simulink model "s_c_nbe_m32k"  (R2016b)
settings: Solver=VariableStepDiscrete  StartTime=0.0  StopTime=2^(fft_stages)*10  RelTol=1e-3
undefined symbols (not defined in the file or in its folder): fft_stages, n_taps, output_bits, xengbits
undefined symbols (not defined in the file): Coeffs, pfb_coeff_gen_calc
libraries: xbsIndex_r4 x12104, xps_library x3, casper_library_delays x2, casper_library_misc x1
(part 21 of 104)

== system s_c_nbe_m32k/DDC/dec_fir_async ==
  sync_in : Inport
  dv_in : Inport  Port=2
  real1 : Inport  Port=3
  imag1 : Inport  Port=4
  real2 : Inport  Port=5
  imag2 : Inport  Port=6
  real3 : Inport  Port=7
  imag3 : Inport  Port=8
  real4 : Inport  Port=9
  imag4 : Inport  Port=10
  real5 : Inport  Port=11
  imag5 : Inport  Port=12
  real6 : Inport  Port=13
  imag6 : Inport  Port=14
  real7 : Inport  Port=15
  imag7 : Inport  Port=16
  real8 : Inport  Port=17
  imag8 : Inport  Port=18
  convert1 : xbsIndex_r4/Convert  gui_display_data_type=Fixed-point  arith_type="Signed  (2's comp)"  n_bits=25  bin_pt=24  float_type=Single  exp_bits=8  fraction_bits=24  quantization="Round  (unbiased: +/- Inf)"  overflow=Wrap  en=off  latency=2  pipeline=off  dbl_ovrd=off  block_type=convert
  convert2 : xbsIndex_r4/Convert  gui_display_data_type=Fixed-point  arith_type="Signed  (2's comp)"  n_bits=25  bin_pt=24  float_type=Single  exp_bits=8  fraction_bits=24  quantization="Round  (unbiased: +/- Inf)"  overflow=Wrap  en=off  latency=2  pipeline=off  dbl_ovrd=off  block_type=convert
  dv_delay : xbsIndex_r4/Delay  rst=off  infoeditControl=Selection of Reset will increase slice count due to use of real FFs and instead of SRLs  en=off  latency=13  reg_retiming=off  dbl_ovrd=off  block_type=delay
      settings: infoedit=Hardware notes: A delay line is a chain, each link of which is an SRL16 or SRL32 followed by a flip-flop.
  fir_col_async1 : Subsystem  AncestorBlock=casper_library_downconverter/fir_col_async  mask(fir_col_async){n_inputs=8, coeff=[0.00099428  0.00087065  0.00071858  0.00055833  0.00040616  0.00027356  0.00016693   0.0001122], add_latency=1, mult_latency=2, coeff_bit_width=25, coeff_bin_pt=24, first_stage_hdl=on, adder_imp=DSP48, async=on, bus_input=off, input_width=0, input_bp=0, input_type=Signed, dbl=on}
      mask prompts: n_inputs "Inputs"; coeff "Coefficients"; add_latency "Add latency"; mult_latency "Mult Latency"; coeff_bit_width "Coefficient bit width"; coeff_bin_pt "Coefficient binary point"; first_stage_hdl "Implement first stage of adder trees on output as behavioural HDL"; adder_imp "Adder implementation"; async "Asynchronous ops"; bus_input "Bus input"; input_width "Input bitwidth"; input_bp "Input binary point"; input_type "Input datatype"; dbl "Double col"
      mask init:
      | fir_col_async_init(gcb);
      mask Help: eval('xlWeb(''http://casper.berkeley.edu/wiki/Fir_col'')')
      mask TypeOptions adder_imp: Behavioral | Fabric | DSP48
      mask Callback bus_input:
      | onoff = get_param(gcb, 'bus_input');
      | set_param_state(gcb, 'input_width', onoff)
      | set_param_state(gcb, 'input_bp', onoff)
      | set_param_state(gcb, 'input_type', onoff)
      mask TypeOptions input_type: Signed | Unsigned
  fir_col_async10 : Subsystem  AncestorBlock=casper_library_downconverter/fir_col_async  mask(fir_col_async){n_inputs=8, coeff=[0.0010344  0.00087109  0.00057317  0.00018922 -0.00021959 -0.00058921  -0.0008627  -0.0009989], add_latency=1, mult_latency=2, coeff_bit_width=25, coeff_bin_pt=24, first_stage_hdl=on, adder_imp=DSP48, async=on, bus_input=off, input_width=0, input_bp=0, input_type=Signed, dbl=on}
      mask prompts: n_inputs "Inputs"; coeff "Coefficients"; add_latency "Add latency"; mult_latency "Mult Latency"; coeff_bit_width "Coefficient bit width"; coeff_bin_pt "Coefficient binary point"; first_stage_hdl "Implement first stage of adder trees on output as behavioural HDL"; adder_imp "Adder implementation"; async "Asynchronous ops"; bus_input "Bus input"; input_width "Input bitwidth"; input_bp "Input binary point"; input_type "Input datatype"; dbl "Double col"
      mask init:
      | fir_col_async_init(gcb);
      mask Help: eval('xlWeb(''http://casper.berkeley.edu/wiki/Fir_col'')')
      mask TypeOptions adder_imp: Behavioral | Fabric | DSP48
      mask Callback bus_input:
      | onoff = get_param(gcb, 'bus_input');
      | set_param_state(gcb, 'input_width', onoff)
      | set_param_state(gcb, 'input_bp', onoff)
      | set_param_state(gcb, 'input_type', onoff)
      mask TypeOptions input_type: Signed | Unsigned
  fir_col_async11 : Subsystem  AncestorBlock=casper_library_downconverter/fir_col_async  mask(fir_col_async){n_inputs=8, coeff=[-0.0011284 -0.00097771 -0.00067706 -0.00027629     0.00016  0.00056292  0.00087004    0.001035], add_latency=1, mult_latency=2, coeff_bit_width=25, coeff_bin_pt=24, first_stage_hdl=on, adder_imp=DSP48, async=on, bus_input=off, input_width=0, input_bp=0, input_type=Signed, dbl=on}
      mask prompts: n_inputs "Inputs"; coeff "Coefficients"; add_latency "Add latency"; mult_latency "Mult Latency"; coeff_bit_width "Coefficient bit width"; coeff_bin_pt "Coefficient binary point"; first_stage_hdl "Implement first stage of adder trees on output as behavioural HDL"; adder_imp "Adder implementation"; async "Asynchronous ops"; bus_input "Bus input"; input_width "Input bitwidth"; input_bp "Input binary point"; input_type "Input datatype"; dbl "Double col"
      mask init:
      | fir_col_async_init(gcb);
      mask Help: eval('xlWeb(''http://casper.berkeley.edu/wiki/Fir_col'')')
      mask TypeOptions adder_imp: Behavioral | Fabric | DSP48
      mask Callback bus_input:
      | onoff = get_param(gcb, 'bus_input');
      | set_param_state(gcb, 'input_width', onoff)
      | set_param_state(gcb, 'input_bp', onoff)
      | set_param_state(gcb, 'input_type', onoff)
      mask TypeOptions input_type: Signed | Unsigned
  fir_col_async12 : Subsystem  AncestorBlock=casper_library_downconverter/fir_col_async  mask(fir_col_async){n_inputs=8, coeff=[0.0012278   0.0010924  0.00078831  0.00036676 -0.00010386  -0.0005489 -0.00089924   -0.001102], add_latency=1, mult_latency=2, coeff_bit_width=25, coeff_bin_pt=24, first_stage_hdl=on, adder_imp=DSP48, async=on, bus_input=off, input_width=0, input_bp=0, input_type=Signed, dbl=on}
      mask prompts: n_inputs "Inputs"; coeff "Coefficients"; add_latency "Add latency"; mult_latency "Mult Latency"; coeff_bit_width "Coefficient bit width"; coeff_bin_pt "Coefficient binary point"; first_stage_hdl "Implement first stage of adder trees on output as behavioural HDL"; adder_imp "Adder implementation"; async "Asynchronous ops"; bus_input "Bus input"; input_width "Input bitwidth"; input_bp "Input binary point"; input_type "Input datatype"; dbl "Double col"
      mask init:
      | fir_col_async_init(gcb);
      mask Help: eval('xlWeb(''http://casper.berkeley.edu/wiki/Fir_col'')')
      mask TypeOptions adder_imp: Behavioral | Fabric | DSP48
      mask Callback bus_input:
      | onoff = get_param(gcb, 'bus_input');
      | set_param_state(gcb, 'input_width', onoff)
      | set_param_state(gcb, 'input_bp', onoff)
      | set_param_state(gcb, 'input_type', onoff)
      mask TypeOptions input_type: Signed | Unsigned
  fir_col_async13 : Subsystem  AncestorBlock=casper_library_downconverter/fir_col_async  mask(fir_col_async){n_inputs=8, coeff=[-0.0013452  -0.0012298 -0.00092426 -0.00048074  2.8225e-05  0.00052148  0.00092209   0.0011693], add_latency=1, mult_latency=2, coeff_bit_width=25, coeff_bin_pt=24, first_stage_hdl=on, adder_imp=DSP48, async=on, bus_input=off, input_width=0, input_bp=0, input_type=Signed, dbl=on}
      mask prompts: n_inputs "Inputs"; coeff "Coefficients"; add_latency "Add latency"; mult_latency "Mult Latency"; coeff_bit_width "Coefficient bit width"; coeff_bin_pt "Coefficient binary point"; first_stage_hdl "Implement first stage of adder trees on output as behavioural HDL"; adder_imp "Adder implementation"; async "Asynchronous ops"; bus_input "Bus input"; input_width "Input bitwidth"; input_bp "Input binary point"; input_type "Input datatype"; dbl "Double col"
      mask init:
      | fir_col_async_init(gcb);
      mask Help: eval('xlWeb(''http://casper.berkeley.edu/wiki/Fir_col'')')
      mask TypeOptions adder_imp: Behavioral | Fabric | DSP48
      mask Callback bus_input:
      | onoff = get_param(gcb, 'bus_input');
      | set_param_state(gcb, 'input_width', onoff)
      | set_param_state(gcb, 'input_bp', onoff)
      | set_param_state(gcb, 'input_type', onoff)
      mask TypeOptions input_type: Signed | Unsigned
  fir_col_async14 : Subsystem  AncestorBlock=casper_library_downconverter/fir_col_async  mask(fir_col_async){n_inputs=8, coeff=[0.0014712   0.0013813   0.0010768  0.00061055  5.9232e-05 -0.00048875 -0.00094762  -0.0012475], add_latency=1, mult_latency=2, coeff_bit_width=25, coeff_bin_pt=24, first_stage_hdl=on, adder_imp=DSP48, async=on, bus_input=off, input_width=0, input_bp=0, input_type=Signed, dbl=on}
      mask prompts: n_inputs "Inputs"; coeff "Coefficients"; add_latency "Add latency"; mult_latency "Mult Latency"; coeff_bit_width "Coefficient bit width"; coeff_bin_pt "Coefficient binary point"; first_stage_hdl "Implement first stage of adder trees on output as behavioural HDL"; adder_imp "Adder implementation"; async "Asynchronous ops"; bus_input "Bus input"; input_width "Input bitwidth"; input_bp "Input binary point"; input_type "Input datatype"; dbl "Double col"
      mask init:
      | fir_col_async_init(gcb);
      mask Help: eval('xlWeb(''http://casper.berkeley.edu/wiki/Fir_col'')')
      mask TypeOptions adder_imp: Behavioral | Fabric | DSP48
      mask Callback bus_input:
      | onoff = get_param(gcb, 'bus_input');
      | set_param_state(gcb, 'input_width', onoff)
      | set_param_state(gcb, 'input_bp', onoff)
      | set_param_state(gcb, 'input_type', onoff)
      mask TypeOptions input_type: Signed | Unsigned
  fir_col_async15 : Subsystem  AncestorBlock=casper_library_downconverter/fir_col_async  mask(fir_col_async){n_inputs=8, coeff=[-0.0016083  -0.0015511  -0.0012519 -0.00076349 -0.00016703  0.00044142   0.0009662    0.001327], add_latency=1, mult_latency=2, coeff_bit_width=25, coeff_bin_pt=24, first_stage_hdl=on, adder_imp=DSP48, async=on, bus_input=off, input_width=0, input_bp=0, input_type=Signed, dbl=on}
      mask prompts: n_inputs "Inputs"; coeff "Coefficients"; add_latency "Add latency"; mult_latency "Mult Latency"; coeff_bit_width "Coefficient bit width"; coeff_bin_pt "Coefficient binary point"; first_stage_hdl "Implement first stage of adder trees on output as behavioural HDL"; adder_imp "Adder implementation"; async "Asynchronous ops"; bus_input "Bus input"; input_width "Input bitwidth"; input_bp "Input binary point"; input_type "Input datatype"; dbl "Double col"
      mask init:
      | fir_col_async_init(gcb);
      mask Help: eval('xlWeb(''http://casper.berkeley.edu/wiki/Fir_col'')')
      mask TypeOptions adder_imp: Behavioral | Fabric | DSP48
      mask Callback bus_input:
      | onoff = get_param(gcb, 'bus_input');
      | set_param_state(gcb, 'input_width', onoff)
      | set_param_state(gcb, 'input_bp', onoff)
      | set_param_state(gcb, 'input_type', onoff)
      mask TypeOptions input_type: Signed | Unsigned
  fir_col_async16 : Subsystem  AncestorBlock=casper_library_downconverter/fir_col_async  mask(fir_col_async){n_inputs=8, coeff=[0.0017552    0.001739   0.0014503  0.00094121    0.000297   -0.000378 -0.00097719  -0.0014085], add_latency=1, mult_latency=2, coeff_bit_width=25, coeff_bin_pt=24, first_stage_hdl=on, adder_imp=DSP48, async=on, bus_input=off, input_width=0, input_bp=0, input_type=Signed, dbl=on}
      mask prompts: n_inputs "Inputs"; coeff "Coefficients"; add_latency "Add latency"; mult_latency "Mult Latency"; coeff_bit_width "Coefficient bit width"; coeff_bin_pt "Coefficient binary point"; first_stage_hdl "Implement first stage of adder trees on output as behavioural HDL"; adder_imp "Adder implementation"; async "Asynchronous ops"; bus_input "Bus input"; input_width "Input bitwidth"; input_bp "Input binary point"; input_type "Input datatype"; dbl "Double col"
      mask init:
      | fir_col_async_init(gcb);
      mask Help: eval('xlWeb(''http://casper.berkeley.edu/wiki/Fir_col'')')
      mask TypeOptions adder_imp: Behavioral | Fabric | DSP48
      mask Callback bus_input:
      | onoff = get_param(gcb, 'bus_input');
      | set_param_state(gcb, 'input_width', onoff)
      | set_param_state(gcb, 'input_bp', onoff)
      | set_param_state(gcb, 'input_type', onoff)
      mask TypeOptions input_type: Signed | Unsigned
  fir_col_async17 : Subsystem  AncestorBlock=casper_library_downconverter/fir_col_async  mask(fir_col_async){n_inputs=8, coeff=[-0.0019109  -0.0019456  -0.0016741  -0.0011468 -0.00045281  0.00029476  0.00097735   0.0014895], add_latency=1, mult_latency=2, coeff_bit_width=25, coeff_bin_pt=24, first_stage_hdl=on, adder_imp=DSP48, async=on, bus_input=off, input_width=0, input_bp=0, input_type=Signed, dbl=on}
      mask prompts: n_inputs "Inputs"; coeff "Coefficients"; add_latency "Add latency"; mult_latency "Mult Latency"; coeff_bit_width "Coefficient bit width"; coeff_bin_pt "Coefficient binary point"; first_stage_hdl "Implement first stage of adder trees on output as behavioural HDL"; adder_imp "Adder implementation"; async "Asynchronous ops"; bus_input "Bus input"; input_width "Input bitwidth"; input_bp "Input binary point"; input_type "Input datatype"; dbl "Double col"
      mask init:
      | fir_col_async_init(gcb);
      mask Help: eval('xlWeb(''http://casper.berkeley.edu/wiki/Fir_col'')')
      mask TypeOptions adder_imp: Behavioral | Fabric | DSP48
      mask Callback bus_input:
      | onoff = get_param(gcb, 'bus_input');
      | set_param_state(gcb, 'input_width', onoff)
      | set_param_state(gcb, 'input_bp', onoff)
      | set_param_state(gcb, 'input_type', onoff)
      mask TypeOptions input_type: Signed | Unsigned
  fir_col_async18 : Subsystem  AncestorBlock=casper_library_downconverter/fir_col_async  mask(fir_col_async){n_inputs=8, coeff=[0.0020752   0.0021728   0.0019267   0.0013847  0.00063944 -0.00018695 -0.00096274  -0.0015675], add_latency=1, mult_latency=2, coeff_bit_width=25, coeff_bin_pt=24, first_stage_hdl=on, adder_imp=DSP48, async=on, bus_input=off, input_width=0, input_bp=0, input_type=Signed, dbl=on}
      mask prompts: n_inputs "Inputs"; coeff "Coefficients"; add_latency "Add latency"; mult_latency "Mult Latency"; coeff_bit_width "Coefficient bit width"; coeff_bin_pt "Coefficient binary point"; first_stage_hdl "Implement first stage of adder trees on output as behavioural HDL"; adder_imp "Adder implementation"; async "Asynchronous ops"; bus_input "Bus input"; input_width "Input bitwidth"; input_bp "Input binary point"; input_type "Input datatype"; dbl "Double col"
      mask init:
      | fir_col_async_init(gcb);
      mask Help: eval('xlWeb(''http://casper.berkeley.edu/wiki/Fir_col'')')
      mask TypeOptions adder_imp: Behavioral | Fabric | DSP48
      mask Callback bus_input:
      | onoff = get_param(gcb, 'bus_input');
      | set_param_state(gcb, 'input_width', onoff)
      | set_param_state(gcb, 'input_bp', onoff)
      | set_param_state(gcb, 'input_type', onoff)
      mask TypeOptions input_type: Signed | Unsigned
  fir_col_async19 : Subsystem  AncestorBlock=casper_library_downconverter/fir_col_async  mask(fir_col_async){n_inputs=8, coeff=[-0.0022479  -0.0024222  -0.0022116  -0.0016596 -0.00086187  4.9984e-05  0.00092987   0.0016406], add_latency=1, mult_latency=2, coeff_bit_width=25, coeff_bin_pt=24, first_stage_hdl=on, adder_imp=DSP48, async=on, bus_input=off, input_width=0, input_bp=0, input_type=Signed, dbl=on}
      mask prompts: n_inputs "Inputs"; coeff "Coefficients"; add_latency "Add latency"; mult_latency "Mult Latency"; coeff_bit_width "Coefficient bit width"; coeff_bin_pt "Coefficient binary point"; first_stage_hdl "Implement first stage of adder trees on output as behavioural HDL"; adder_imp "Adder implementation"; async "Asynchronous ops"; bus_input "Bus input"; input_width "Input bitwidth"; input_bp "Input binary point"; input_type "Input datatype"; dbl "Double col"
      mask init:
      | fir_col_async_init(gcb);
      mask Help: eval('xlWeb(''http://casper.berkeley.edu/wiki/Fir_col'')')
      mask TypeOptions adder_imp: Behavioral | Fabric | DSP48
      mask Callback bus_input:
      | onoff = get_param(gcb, 'bus_input');
      | set_param_state(gcb, 'input_width', onoff)
      | set_param_state(gcb, 'input_bp', onoff)
      | set_param_state(gcb, 'input_type', onoff)
      mask TypeOptions input_type: Signed | Unsigned
  fir_col_async2 : Subsystem  AncestorBlock=casper_library_downconverter/fir_col_async  mask(fir_col_async){n_inputs=8, coeff=[-0.0011022 -0.00050891  1.6603e-05  0.00044686  0.00076606  0.00097017   0.0010656   0.0010669], add_latency=1, mult_latency=2, coeff_bit_width=25, coeff_bin_pt=24, first_stage_hdl=on, adder_imp=DSP48, async=on, bus_input=off, input_width=0, input_bp=0, input_type=Signed, dbl=on}
      mask prompts: n_inputs "Inputs"; coeff "Coefficients"; add_latency "Add latency"; mult_latency "Mult Latency"; coeff_bit_width "Coefficient bit width"; coeff_bin_pt "Coefficient binary point"; first_stage_hdl "Implement first stage of adder trees on output as behavioural HDL"; adder_imp "Adder implementation"; async "Asynchronous ops"; bus_input "Bus input"; input_width "Input bitwidth"; input_bp "Input binary point"; input_type "Input datatype"; dbl "Double col"
      mask init:
      | fir_col_async_init(gcb);
      mask Help: eval('xlWeb(''http://casper.berkeley.edu/wiki/Fir_col'')')
      mask TypeOptions adder_imp: Behavioral | Fabric | DSP48
      mask Callback bus_input:
      | onoff = get_param(gcb, 'bus_input');
      | set_param_state(gcb, 'input_width', onoff)
      | set_param_state(gcb, 'input_bp', onoff)
      | set_param_state(gcb, 'input_type', onoff)
      mask TypeOptions input_type: Signed | Unsigned
  fir_col_async20 : Subsystem  AncestorBlock=casper_library_downconverter/fir_col_async  mask(fir_col_async){n_inputs=8, coeff=[0.0024274   0.0026955   0.0025329   0.0019771   0.0011263  0.00012192 -0.00087426  -0.0017062], add_latency=1, mult_latency=2, coeff_bit_width=25, coeff_bin_pt=24, first_stage_hdl=on, adder_imp=DSP48, async=on, bus_input=off, input_width=0, input_bp=0, input_type=Signed, dbl=on}
      mask prompts: n_inputs "Inputs"; coeff "Coefficients"; add_latency "Add latency"; mult_latency "Mult Latency"; coeff_bit_width "Coefficient bit width"; coeff_bin_pt "Coefficient binary point"; first_stage_hdl "Implement first stage of adder trees on output as behavioural HDL"; adder_imp "Adder implementation"; async "Asynchronous ops"; bus_input "Bus input"; input_width "Input bitwidth"; input_bp "Input binary point"; input_type "Input datatype"; dbl "Double col"
      mask init:
      | fir_col_async_init(gcb);
      mask Help: eval('xlWeb(''http://casper.berkeley.edu/wiki/Fir_col'')')
      mask TypeOptions adder_imp: Behavioral | Fabric | DSP48
      mask Callback bus_input:
      | onoff = get_param(gcb, 'bus_input');
      | set_param_state(gcb, 'input_width', onoff)
      | set_param_state(gcb, 'input_bp', onoff)
      | set_param_state(gcb, 'input_type', onoff)
      mask TypeOptions input_type: Signed | Unsigned
  fir_col_async21 : Subsystem  AncestorBlock=casper_library_downconverter/fir_col_async  mask(fir_col_async){n_inputs=8, coeff=[-0.0026176  -0.0029997     -0.0029  -0.0023482  -0.0014437 -0.00033851  0.00078838   0.0017597], add_latency=1, mult_latency=2, coeff_bit_width=25, coeff_bin_pt=24, first_stage_hdl=on, adder_imp=DSP48, async=on, bus_input=off, input_width=0, input_bp=0, input_type=Signed, dbl=on}
      mask prompts: n_inputs "Inputs"; coeff "Coefficients"; add_latency "Add latency"; mult_latency "Mult Latency"; coeff_bit_width "Coefficient bit width"; coeff_bin_pt "Coefficient binary point"; first_stage_hdl "Implement first stage of adder trees on output as behavioural HDL"; adder_imp "Adder implementation"; async "Asynchronous ops"; bus_input "Bus input"; input_width "Input bitwidth"; input_bp "Input binary point"; input_type "Input datatype"; dbl "Double col"
      mask init:
      | fir_col_async_init(gcb);
      mask Help: eval('xlWeb(''http://casper.berkeley.edu/wiki/Fir_col'')')
      mask TypeOptions adder_imp: Behavioral | Fabric | DSP48
      mask Callback bus_input:
      | onoff = get_param(gcb, 'bus_input');
      | set_param_state(gcb, 'input_width', onoff)
      | set_param_state(gcb, 'input_bp', onoff)
      | set_param_state(gcb, 'input_type', onoff)
      mask TypeOptions input_type: Signed | Unsigned
  fir_col_async22 : Subsystem  AncestorBlock=casper_library_downconverter/fir_col_async  mask(fir_col_async){n_inputs=8, coeff=[0.0028147   0.0033361    0.003318   0.0027798   0.0018215  0.00060595 -0.00066876   -0.001801], add_latency=1, mult_latency=2, coeff_bit_width=25, coeff_bin_pt=24, first_stage_hdl=on, adder_imp=DSP48, async=on, bus_input=off, input_width=0, input_bp=0, input_type=Signed, dbl=on}
      mask prompts: n_inputs "Inputs"; coeff "Coefficients"; add_latency "Add latency"; mult_latency "Mult Latency"; coeff_bit_width "Coefficient bit width"; coeff_bin_pt "Coefficient binary point"; first_stage_hdl "Implement first stage of adder trees on output as behavioural HDL"; adder_imp "Adder implementation"; async "Asynchronous ops"; bus_input "Bus input"; input_width "Input bitwidth"; input_bp "Input binary point"; input_type "Input datatype"; dbl "Double col"
      mask init:
      | fir_col_async_init(gcb);
      mask Help: eval('xlWeb(''http://casper.berkeley.edu/wiki/Fir_col'')')
      mask TypeOptions adder_imp: Behavioral | Fabric | DSP48
      mask Callback bus_input:
      | onoff = get_param(gcb, 'bus_input');
      | set_param_state(gcb, 'input_width', onoff)
      | set_param_state(gcb, 'input_bp', onoff)
      | set_param_state(gcb, 'input_type', onoff)
      mask TypeOptions input_type: Signed | Unsigned
  fir_col_async23 : Subsystem  AncestorBlock=casper_library_downconverter/fir_col_async  mask(fir_col_async){n_inputs=8, coeff=[-0.0030251  -0.0037182  -0.0038056  -0.0032934   -0.002281 -0.00094296   0.0005009   0.0018211], add_latency=1, mult_latency=2, coeff_bit_width=25, coeff_bin_pt=24, first_stage_hdl=on, adder_imp=DSP48, async=on, bus_input=off, input_width=0, input_bp=0, input_type=Signed, dbl=on}
      mask prompts: n_inputs "Inputs"; coeff "Coefficients"; add_latency "Add latency"; mult_latency "Mult Latency"; coeff_bit_width "Coefficient bit width"; coeff_bin_pt "Coefficient binary point"; first_stage_hdl "Implement first stage of adder trees on output as behavioural HDL"; adder_imp "Adder implementation"; async "Asynchronous ops"; bus_input "Bus input"; input_width "Input bitwidth"; input_bp "Input binary point"; input_type "Input datatype"; dbl "Double col"
      mask init:
      | fir_col_async_init(gcb);
      mask Help: eval('xlWeb(''http://casper.berkeley.edu/wiki/Fir_col'')')
      mask TypeOptions adder_imp: Behavioral | Fabric | DSP48
      mask Callback bus_input:
      | onoff = get_param(gcb, 'bus_input');
      | set_param_state(gcb, 'input_width', onoff)
      | set_param_state(gcb, 'input_bp', onoff)
      | set_param_state(gcb, 'input_type', onoff)
      mask TypeOptions input_type: Signed | Unsigned
  fir_col_async24 : Subsystem  AncestorBlock=casper_library_downconverter/fir_col_async  mask(fir_col_async){n_inputs=8, coeff=[0.0032547   0.0041608   0.0043834   0.0039118   0.0028437   0.0013665 -0.00027482  -0.0018181], add_latency=1, mult_latency=2, coeff_bit_width=25, coeff_bin_pt=24, first_stage_hdl=on, adder_imp=DSP48, async=on, bus_input=off, input_width=0, input_bp=0, input_type=Signed, dbl=on}
      mask prompts: n_inputs "Inputs"; coeff "Coefficients"; add_latency "Add latency"; mult_latency "Mult Latency"; coeff_bit_width "Coefficient bit width"; coeff_bin_pt "Coefficient binary point"; first_stage_hdl "Implement first stage of adder trees on output as behavioural HDL"; adder_imp "Adder implementation"; async "Asynchronous ops"; bus_input "Bus input"; input_width "Input bitwidth"; input_bp "Input binary point"; input_type "Input datatype"; dbl "Double col"
      mask init:
      | fir_col_async_init(gcb);
      mask Help: eval('xlWeb(''http://casper.berkeley.edu/wiki/Fir_col'')')
      mask TypeOptions adder_imp: Behavioral | Fabric | DSP48
      mask Callback bus_input:
      | onoff = get_param(gcb, 'bus_input');
      | set_param_state(gcb, 'input_width', onoff)
      | set_param_state(gcb, 'input_bp', onoff)
      | set_param_state(gcb, 'input_type', onoff)
      mask TypeOptions input_type: Signed | Unsigned
  fir_col_async25 : Subsystem  AncestorBlock=casper_library_downconverter/fir_col_async  mask(fir_col_async){n_inputs=8, coeff=[-0.0035051  -0.0046808   -0.005079  -0.0046673  -0.0035408   -0.001902 -2.5483e-05    0.001787], add_latency=1, mult_latency=2, coeff_bit_width=25, coeff_bin_pt=24, first_stage_hdl=on, adder_imp=DSP48, async=on, bus_input=off, input_width=0, input_bp=0, input_type=Signed, dbl=on}
      mask prompts: n_inputs "Inputs"; coeff "Coefficients"; add_latency "Add latency"; mult_latency "Mult Latency"; coeff_bit_width "Coefficient bit width"; coeff_bin_pt "Coefficient binary point"; first_stage_hdl "Implement first stage of adder trees on output as behavioural HDL"; adder_imp "Adder implementation"; async "Asynchronous ops"; bus_input "Bus input"; input_width "Input bitwidth"; input_bp "Input binary point"; input_type "Input datatype"; dbl "Double col"
      mask init:
      | fir_col_async_init(gcb);
      mask Help: eval('xlWeb(''http://casper.berkeley.edu/wiki/Fir_col'')')
      mask TypeOptions adder_imp: Behavioral | Fabric | DSP48
      mask Callback bus_input:
      | onoff = get_param(gcb, 'bus_input');
      | set_param_state(gcb, 'input_width', onoff)
      | set_param_state(gcb, 'input_bp', onoff)
      | set_param_state(gcb, 'input_type', onoff)
      mask TypeOptions input_type: Signed | Unsigned
  fir_col_async26 : Subsystem  AncestorBlock=casper_library_downconverter/fir_col_async  mask(fir_col_async){n_inputs=8, coeff=[0.0037941   0.0053211   0.0059514   0.0056257   0.0044352   0.0026011  0.00043547  -0.0017112], add_latency=1, mult_latency=2, coeff_bit_width=25, coeff_bin_pt=24, first_stage_hdl=on, adder_imp=DSP48, async=on, bus_input=off, input_width=0, input_bp=0, input_type=Signed, dbl=on}
      mask prompts: n_inputs "Inputs"; coeff "Coefficients"; add_latency "Add latency"; mult_latency "Mult Latency"; coeff_bit_width "Coefficient bit width"; coeff_bin_pt "Coefficient binary point"; first_stage_hdl "Implement first stage of adder trees on output as behavioural HDL"; adder_imp "Adder implementation"; async "Asynchronous ops"; bus_input "Bus input"; input_width "Input bitwidth"; input_bp "Input binary point"; input_type "Input datatype"; dbl "Double col"
      mask init:
      | fir_col_async_init(gcb);
      mask Help: eval('xlWeb(''http://casper.berkeley.edu/wiki/Fir_col'')')
      mask TypeOptions adder_imp: Behavioral | Fabric | DSP48
      mask Callback bus_input:
      | onoff = get_param(gcb, 'bus_input');
      | set_param_state(gcb, 'input_width', onoff)
      | set_param_state(gcb, 'input_bp', onoff)
      | set_param_state(gcb, 'input_type', onoff)
      mask TypeOptions input_type: Signed | Unsigned
  fir_col_async27 : Subsystem  AncestorBlock=casper_library_downconverter/fir_col_async  mask(fir_col_async){n_inputs=8, coeff=[-0.0041452  -0.0061485  -0.0070947  -0.0068901  -0.0056225   -0.003539  -0.0010009   0.0015775], add_latency=1, mult_latency=2, coeff_bit_width=25, coeff_bin_pt=24, first_stage_hdl=on, adder_imp=DSP48, async=on, bus_input=off, input_width=0, input_bp=0, input_type=Signed, dbl=on}
      mask prompts: n_inputs "Inputs"; coeff "Coefficients"; add_latency "Add latency"; mult_latency "Mult Latency"; coeff_bit_width "Coefficient bit width"; coeff_bin_pt "Coefficient binary point"; first_stage_hdl "Implement first stage of adder trees on output as behavioural HDL"; adder_imp "Adder implementation"; async "Asynchronous ops"; bus_input "Bus input"; input_width "Input bitwidth"; input_bp "Input binary point"; input_type "Input datatype"; dbl "Double col"
      mask init:
      | fir_col_async_init(gcb);
      mask Help: eval('xlWeb(''http://casper.berkeley.edu/wiki/Fir_col'')')
      mask TypeOptions adder_imp: Behavioral | Fabric | DSP48
      mask Callback bus_input:
      | onoff = get_param(gcb, 'bus_input');
      | set_param_state(gcb, 'input_width', onoff)
      | set_param_state(gcb, 'input_bp', onoff)
      | set_param_state(gcb, 'input_type', onoff)
      mask TypeOptions input_type: Signed | Unsigned
  fir_col_async28 : Subsystem  AncestorBlock=casper_library_downconverter/fir_col_async  mask(fir_col_async){n_inputs=8, coeff=[0.0046135   0.0073018   0.0086977   0.0086643   0.0072901   0.0048624   0.0018131  -0.0013542], add_latency=1, mult_latency=2, coeff_bit_width=25, coeff_bin_pt=24, first_stage_hdl=on, adder_imp=DSP48, async=on, bus_input=off, input_width=0, input_bp=0, input_type=Signed, dbl=on}
      mask prompts: n_inputs "Inputs"; coeff "Coefficients"; add_latency "Add latency"; mult_latency "Mult Latency"; coeff_bit_width "Coefficient bit width"; coeff_bin_pt "Coefficient binary point"; first_stage_hdl "Implement first stage of adder trees on output as behavioural HDL"; adder_imp "Adder implementation"; async "Asynchronous ops"; bus_input "Bus input"; input_width "Input bitwidth"; input_bp "Input binary point"; input_type "Input datatype"; dbl "Double col"
      mask init:
      | fir_col_async_init(gcb);
      mask Help: eval('xlWeb(''http://casper.berkeley.edu/wiki/Fir_col'')')
      mask TypeOptions adder_imp: Behavioral | Fabric | DSP48
      mask Callback bus_input:
      | onoff = get_param(gcb, 'bus_input');
      | set_param_state(gcb, 'input_width', onoff)
      | set_param_state(gcb, 'input_bp', onoff)
      | set_param_state(gcb, 'input_type', onoff)
      mask TypeOptions input_type: Signed | Unsigned
  fir_col_async29 : Subsystem  AncestorBlock=casper_library_downconverter/fir_col_async  mask(fir_col_async){n_inputs=8, coeff=[-0.0053149  -0.0090842   -0.011168   -0.011381  -0.0098267   -0.006868  -0.0030507  0.00098655], add_latency=1, mult_latency=2, coeff_bit_width=25, coeff_bin_pt=24, first_stage_hdl=on, adder_imp=DSP48, async=on, bus_input=off, input_width=0, input_bp=0, input_type=Signed, dbl=on}
      mask prompts: n_inputs "Inputs"; coeff "Coefficients"; add_latency "Add latency"; mult_latency "Mult Latency"; coeff_bit_width "Coefficient bit width"; coeff_bin_pt "Coefficient binary point"; first_stage_hdl "Implement first stage of adder trees on output as behavioural HDL"; adder_imp "Adder implementation"; async "Asynchronous ops"; bus_input "Bus input"; input_width "Input bitwidth"; input_bp "Input binary point"; input_type "Input datatype"; dbl "Double col"
      mask init:
      | fir_col_async_init(gcb);
      mask Help: eval('xlWeb(''http://casper.berkeley.edu/wiki/Fir_col'')')
      mask TypeOptions adder_imp: Behavioral | Fabric | DSP48
      mask Callback bus_input:
      | onoff = get_param(gcb, 'bus_input');
      | set_param_state(gcb, 'input_width', onoff)
      | set_param_state(gcb, 'input_bp', onoff)
      | set_param_state(gcb, 'input_type', onoff)
      mask TypeOptions input_type: Signed | Unsigned
  fir_col_async3 : Subsystem  AncestorBlock=casper_library_downconverter/fir_col_async  mask(fir_col_async){n_inputs=8, coeff=[-0.0033043   -0.003591  -0.0036874  -0.0035888  -0.0033089  -0.0028768  -0.0023331  -0.0017253], add_latency=1, mult_latency=2, coeff_bit_width=25, coeff_bin_pt=24, first_stage_hdl=on, adder_imp=DSP48, async=on, bus_input=off, input_width=0, input_bp=0, input_type=Signed, dbl=on}
      mask prompts: n_inputs "Inputs"; coeff "Coefficients"; add_latency "Add latency"; mult_latency "Mult Latency"; coeff_bit_width "Coefficient bit width"; coeff_bin_pt "Coefficient binary point"; first_stage_hdl "Implement first stage of adder trees on output as behavioural HDL"; adder_imp "Adder implementation"; async "Asynchronous ops"; bus_input "Bus input"; input_width "Input bitwidth"; input_bp "Input binary point"; input_type "Input datatype"; dbl "Double col"
      mask init:
      | fir_col_async_init(gcb);
      mask Help: eval('xlWeb(''http://casper.berkeley.edu/wiki/Fir_col'')')
      mask TypeOptions adder_imp: Behavioral | Fabric | DSP48
      mask Callback bus_input:
      | onoff = get_param(gcb, 'bus_input');
      | set_param_state(gcb, 'input_width', onoff)
      | set_param_state(gcb, 'input_bp', onoff)
      | set_param_state(gcb, 'input_type', onoff)
      mask TypeOptions input_type: Signed | Unsigned
  fir_col_async30 : Subsystem  AncestorBlock=casper_library_downconverter/fir_col_async  mask(fir_col_async){n_inputs=8, coeff=[0.0066096    0.012373    0.015639    0.016199    0.014246    0.010311   0.0051604 -0.00033145], add_latency=1, mult_latency=2, coeff_bit_width=25, coeff_bin_pt=24, first_stage_hdl=on, adder_imp=DSP48, async=on, bus_input=off, input_width=0, input_bp=0, input_type=Signed, dbl=on}
      mask prompts: n_inputs "Inputs"; coeff "Coefficients"; add_latency "Add latency"; mult_latency "Mult Latency"; coeff_bit_width "Coefficient bit width"; coeff_bin_pt "Coefficient binary point"; first_stage_hdl "Implement first stage of adder trees on output as behavioural HDL"; adder_imp "Adder implementation"; async "Asynchronous ops"; bus_input "Bus input"; input_width "Input bitwidth"; input_bp "Input binary point"; input_type "Input datatype"; dbl "Double col"
      mask init:
      | fir_col_async_init(gcb);
      mask Help: eval('xlWeb(''http://casper.berkeley.edu/wiki/Fir_col'')')
      mask TypeOptions adder_imp: Behavioral | Fabric | DSP48
      mask Callback bus_input:
      | onoff = get_param(gcb, 'bus_input');
      | set_param_state(gcb, 'input_width', onoff)
      | set_param_state(gcb, 'input_bp', onoff)
      | set_param_state(gcb, 'input_type', onoff)
      mask TypeOptions input_type: Signed | Unsigned
  fir_col_async31 : Subsystem  AncestorBlock=casper_library_downconverter/fir_col_async  mask(fir_col_async){n_inputs=8, coeff=[-0.010203    -0.02099   -0.026686   -0.027498   -0.024143   -0.017721   -0.009558  -0.0010299], add_latency=1, mult_latency=2, coeff_bit_width=25, coeff_bin_pt=24, first_stage_hdl=on, adder_imp=DSP48, async=on, bus_input=off, input_width=0, input_bp=0, input_type=Signed, dbl=on}
      mask prompts: n_inputs "Inputs"; coeff "Coefficients"; add_latency "Add latency"; mult_latency "Mult Latency"; coeff_bit_width "Coefficient bit width"; coeff_bin_pt "Coefficient binary point"; first_stage_hdl "Implement first stage of adder trees on output as behavioural HDL"; adder_imp "Adder implementation"; async "Asynchronous ops"; bus_input "Bus input"; input_width "Input bitwidth"; input_bp "Input binary point"; input_type "Input datatype"; dbl "Double col"
      mask init:
      | fir_col_async_init(gcb);
      mask Help: eval('xlWeb(''http://casper.berkeley.edu/wiki/Fir_col'')')
      mask TypeOptions adder_imp: Behavioral | Fabric | DSP48
      mask Callback bus_input:
      | onoff = get_param(gcb, 'bus_input');
      | set_param_state(gcb, 'input_width', onoff)
      | set_param_state(gcb, 'input_bp', onoff)
      | set_param_state(gcb, 'input_type', onoff)
      mask TypeOptions input_type: Signed | Unsigned
  fir_col_async32 : Subsystem  AncestorBlock=casper_library_downconverter/fir_col_async  mask(fir_col_async){n_inputs=8, coeff=[0.12714     0.12037     0.10749    0.089713    0.068703    0.046365    0.024646   0.0053173], add_latency=1, mult_latency=2, coeff_bit_width=25, coeff_bin_pt=24, first_stage_hdl=on, adder_imp=DSP48, async=on, bus_input=off, input_width=0, input_bp=0, input_type=Signed, dbl=on}
      mask prompts: n_inputs "Inputs"; coeff "Coefficients"; add_latency "Add latency"; mult_latency "Mult Latency"; coeff_bit_width "Coefficient bit width"; coeff_bin_pt "Coefficient binary point"; first_stage_hdl "Implement first stage of adder trees on output as behavioural HDL"; adder_imp "Adder implementation"; async "Asynchronous ops"; bus_input "Bus input"; input_width "Input bitwidth"; input_bp "Input binary point"; input_type "Input datatype"; dbl "Double col"
      mask init:
      | fir_col_async_init(gcb);
      mask Help: eval('xlWeb(''http://casper.berkeley.edu/wiki/Fir_col'')')
      mask TypeOptions adder_imp: Behavioral | Fabric | DSP48
      mask Callback bus_input:
      | onoff = get_param(gcb, 'bus_input');
      | set_param_state(gcb, 'input_width', onoff)
      | set_param_state(gcb, 'input_bp', onoff)
      | set_param_state(gcb, 'input_type', onoff)
      mask TypeOptions input_type: Signed | Unsigned
  fir_col_async4 : Subsystem  AncestorBlock=casper_library_downconverter/fir_col_async  mask(fir_col_async){n_inputs=8, coeff=[0.0007137  0.00053475  0.00017744 -0.00033154 -0.00094782  -0.0016146  -0.0022692  -0.0028503], add_latency=1, mult_latency=2, coeff_bit_width=25, coeff_bin_pt=24, first_stage_hdl=on, adder_imp=DSP48, async=on, bus_input=off, input_width=0, input_bp=0, input_type=Signed, dbl=on}
      mask prompts: n_inputs "Inputs"; coeff "Coefficients"; add_latency "Add latency"; mult_latency "Mult Latency"; coeff_bit_width "Coefficient bit width"; coeff_bin_pt "Coefficient binary point"; first_stage_hdl "Implement first stage of adder trees on output as behavioural HDL"; adder_imp "Adder implementation"; async "Asynchronous ops"; bus_input "Bus input"; input_width "Input bitwidth"; input_bp "Input binary point"; input_type "Input datatype"; dbl "Double col"
      mask init:
      | fir_col_async_init(gcb);
      mask Help: eval('xlWeb(''http://casper.berkeley.edu/wiki/Fir_col'')')
      mask TypeOptions adder_imp: Behavioral | Fabric | DSP48
      mask Callback bus_input:
      | onoff = get_param(gcb, 'bus_input');
      | set_param_state(gcb, 'input_width', onoff)
      | set_param_state(gcb, 'input_bp', onoff)
      | set_param_state(gcb, 'input_type', onoff)
      mask TypeOptions input_type: Signed | Unsigned
  fir_col_async5 : Subsystem  AncestorBlock=casper_library_downconverter/fir_col_async  mask(fir_col_async){n_inputs=8, coeff=[-0.0013541  -0.0012105 -0.00093411 -0.00056485 -0.00015653  0.00023015  0.00053552  0.00070862], add_latency=1, mult_latency=2, coeff_bit_width=25, coeff_bin_pt=24, first_stage_hdl=on, adder_imp=DSP48, async=on, bus_input=off, input_width=0, input_bp=0, input_type=Signed, dbl=on}
      mask prompts: n_inputs "Inputs"; coeff "Coefficients"; add_latency "Add latency"; mult_latency "Mult Latency"; coeff_bit_width "Coefficient bit width"; coeff_bin_pt "Coefficient binary point"; first_stage_hdl "Implement first stage of adder trees on output as behavioural HDL"; adder_imp "Adder implementation"; async "Asynchronous ops"; bus_input "Bus input"; input_width "Input bitwidth"; input_bp "Input binary point"; input_type "Input datatype"; dbl "Double col"
      mask init:
      | fir_col_async_init(gcb);
      mask Help: eval('xlWeb(''http://casper.berkeley.edu/wiki/Fir_col'')')
      mask TypeOptions adder_imp: Behavioral | Fabric | DSP48
      mask Callback bus_input:
      | onoff = get_param(gcb, 'bus_input');
      | set_param_state(gcb, 'input_width', onoff)
      | set_param_state(gcb, 'input_bp', onoff)
      | set_param_state(gcb, 'input_type', onoff)
      mask TypeOptions input_type: Signed | Unsigned
  fir_col_async6 : Subsystem  AncestorBlock=casper_library_downconverter/fir_col_async  mask(fir_col_async){n_inputs=8, coeff=[0.00082989  0.00062894  0.00030839 -8.8378e-05  -0.0005068 -0.00088889  -0.0011816  -0.0013441], add_latency=1, mult_latency=2, coeff_bit_width=25, coeff_bin_pt=24, first_stage_hdl=on, adder_imp=DSP48, async=on, bus_input=off, input_width=0, input_bp=0, input_type=Signed, dbl=on}
      mask prompts: n_inputs "Inputs"; coeff "Coefficients"; add_latency "Add latency"; mult_latency "Mult Latency"; coeff_bit_width "Coefficient bit width"; coeff_bin_pt "Coefficient binary point"; first_stage_hdl "Implement first stage of adder trees on output as behavioural HDL"; adder_imp "Adder implementation"; async "Asynchronous ops"; bus_input "Bus input"; input_width "Input bitwidth"; input_bp "Input binary point"; input_type "Input datatype"; dbl "Double col"
      mask init:
      | fir_col_async_init(gcb);
      mask Help: eval('xlWeb(''http://casper.berkeley.edu/wiki/Fir_col'')')
      mask TypeOptions adder_imp: Behavioral | Fabric | DSP48
      mask Callback bus_input:
      | onoff = get_param(gcb, 'bus_input');
      | set_param_state(gcb, 'input_width', onoff)
      | set_param_state(gcb, 'input_bp', onoff)
      | set_param_state(gcb, 'input_type', onoff)
      mask TypeOptions input_type: Signed | Unsigned
  fir_col_async7 : Subsystem  AncestorBlock=casper_library_downconverter/fir_col_async  mask(fir_col_async){n_inputs=8, coeff=[-0.00096395 -0.00078334 -0.00049096 -0.00013198  0.00023829  0.00056265  0.00079052  0.00088532], add_latency=1, mult_latency=2, coeff_bit_width=25, coeff_bin_pt=24, first_stage_hdl=on, adder_imp=DSP48, async=on, bus_input=off, input_width=0, input_bp=0, input_type=Signed, dbl=on}
      mask prompts: n_inputs "Inputs"; coeff "Coefficients"; add_latency "Add latency"; mult_latency "Mult Latency"; coeff_bit_width "Coefficient bit width"; coeff_bin_pt "Coefficient binary point"; first_stage_hdl "Implement first stage of adder trees on output as behavioural HDL"; adder_imp "Adder implementation"; async "Asynchronous ops"; bus_input "Bus input"; input_width "Input bitwidth"; input_bp "Input binary point"; input_type "Input datatype"; dbl "Double col"
      mask init:
      | fir_col_async_init(gcb);
      mask Help: eval('xlWeb(''http://casper.berkeley.edu/wiki/Fir_col'')')
      mask TypeOptions adder_imp: Behavioral | Fabric | DSP48
      mask Callback bus_input:
      | onoff = get_param(gcb, 'bus_input');
      | set_param_state(gcb, 'input_width', onoff)
      | set_param_state(gcb, 'input_bp', onoff)
      | set_param_state(gcb, 'input_type', onoff)
      mask TypeOptions input_type: Signed | Unsigned
  fir_col_async8 : Subsystem  AncestorBlock=casper_library_downconverter/fir_col_async  mask(fir_col_async){n_inputs=8, coeff=[0.00090064  0.00071766  0.00041971  5.2947e-05 -0.00032629 -0.00066016 -0.00089813  -0.0010045], add_latency=1, mult_latency=2, coeff_bit_width=25, coeff_bin_pt=24, first_stage_hdl=on, adder_imp=DSP48, async=on, bus_input=off, input_width=0, input_bp=0, input_type=Signed, dbl=on}
      mask prompts: n_inputs "Inputs"; coeff "Coefficients"; add_latency "Add latency"; mult_latency "Mult Latency"; coeff_bit_width "Coefficient bit width"; coeff_bin_pt "Coefficient binary point"; first_stage_hdl "Implement first stage of adder trees on output as behavioural HDL"; adder_imp "Adder implementation"; async "Asynchronous ops"; bus_input "Bus input"; input_width "Input bitwidth"; input_bp "Input binary point"; input_type "Input datatype"; dbl "Double col"
      mask init:
      | fir_col_async_init(gcb);
      mask Help: eval('xlWeb(''http://casper.berkeley.edu/wiki/Fir_col'')')
      mask TypeOptions adder_imp: Behavioral | Fabric | DSP48
      mask Callback bus_input:
      | onoff = get_param(gcb, 'bus_input');
      | set_param_state(gcb, 'input_width', onoff)
      | set_param_state(gcb, 'input_bp', onoff)
      | set_param_state(gcb, 'input_type', onoff)
      mask TypeOptions input_type: Signed | Unsigned
  fir_col_async9 : Subsystem  AncestorBlock=casper_library_downconverter/fir_col_async  mask(fir_col_async){n_inputs=8, coeff=[-0.00097861 -0.00080718 -0.00051334 -0.00014442  0.00024117  0.00058313  0.00082852  0.00093986], add_latency=1, mult_latency=2, coeff_bit_width=25, coeff_bin_pt=24, first_stage_hdl=on, adder_imp=DSP48, async=on, bus_input=off, input_width=0, input_bp=0, input_type=Signed, dbl=on}
      mask prompts: n_inputs "Inputs"; coeff "Coefficients"; add_latency "Add latency"; mult_latency "Mult Latency"; coeff_bit_width "Coefficient bit width"; coeff_bin_pt "Coefficient binary point"; first_stage_hdl "Implement first stage of adder trees on output as behavioural HDL"; adder_imp "Adder implementation"; async "Asynchronous ops"; bus_input "Bus input"; input_width "Input bitwidth"; input_bp "Input binary point"; input_type "Input datatype"; dbl "Double col"
      mask init:
      | fir_col_async_init(gcb);
      mask Help: eval('xlWeb(''http://casper.berkeley.edu/wiki/Fir_col'')')
      mask TypeOptions adder_imp: Behavioral | Fabric | DSP48
      mask Callback bus_input:
      | onoff = get_param(gcb, 'bus_input');
      | set_param_state(gcb, 'input_width', onoff)
      | set_param_state(gcb, 'input_bp', onoff)
      | set_param_state(gcb, 'input_type', onoff)
      mask TypeOptions input_type: Signed | Unsigned
  imag_sum : Subsystem  AncestorBlock=casper_library_misc/adder_tree  mask(adder_tree){n_inputs=32, latency=1, adder_imp=DSP48, first_stage_hdl=off, floating_point=off, float_type=single, frac_width=0, exp_width=0}
      mask prompts: n_inputs "Number of Inputs"; latency "Add Latency"; adder_imp "Adder implementation"; first_stage_hdl "Use behavioural HDL for first stage of adders"; floating_point "floating point"; float_type "float type"; frac_width "fraction length"; exp_width "exponent length"
      mask help:
      | Sums all inputs using a tree of adds and delays.
      |
      | Number of inputs: The number of inputs to the block to be summed
      | Add latency: The number of clock cycles to perform one addition (affects timing)..
      | Adder implementation: choice of fabric or DSP48E core, or behavioral HDL
      | Use behavioural HDL for first stage of adders: Causes the first stage of adders to be absorbed into DSP blocks if multipliers precede them (Virtex 5). Overrides Adder implementation
      mask init:
      | adder_tree_init(gcb, ...
      |     'n_inputs', n_inputs, ...
      |     'latency', latency, ...
      |     'adder_imp', adder_imp, ...
      |     'floating_point', floating_point, ...
      |     'float_type', float_type, ...
      |     'exp_width', exp_width, ...
      |     'frac_width', frac_width, ...     
      |     'first_stage_hdl', first_stage_hdl);
      settings: AttributesFormatString=latency 5
      mask Help: eval('xlWeb(''http://casper.berkeley.edu/wiki/Adder_tree'')')
      mask TypeOptions adder_imp: Behavioral | Fabric | DSP48
      mask Callback floating_point:
      | onoff = get_param(gcb, 'floating_point');
      | if strcmp(onoff,'on')
      |     enable_fixpt = 'off'
      |     set_param_state(gcb, 'float_type', 'on')
      | 
      |     f_type = get_param(gcb, 'float_type')
      |     if strcmp(f_type,'custom')
      |         set_param_state(gcb, 'exp_width', 'on')
      |         set_param_state(gcb, 'frac_width', 'on')
      |     else
      |         set_param_state(gcb, 'exp_width', 'off')
      |         set_param_state(gcb, 'frac_width', 'off')
      |     end
      | 
      | 
      | else
      |     enable_fixpt = 'on'
      |     set_param_state(gcb, 'float_type', 'off')
      |     set_param_state(gcb, 'exp_width', 'off')
      |     set_param_state(gcb, 'frac_width', 'off')
      | end
      mask TypeOptions float_type: single | custom
      mask Callback float_type:
      | f_type = get_param(gcb, 'float_type')
      | if strcmp(f_type,'custom')
      |     set_param_state(gcb, 'exp_width', 'on')
      |     set_param_state(gcb, 'frac_width', 'on')
      | else
      |     set_param_state(gcb, 'exp_width', 'off')
      |     set_param_state(gcb, 'frac_width', 'off')
      | end
  real_sum : Subsystem  AncestorBlock=casper_library_misc/adder_tree  mask(adder_tree){n_inputs=32, latency=1, adder_imp=DSP48, first_stage_hdl=off, floating_point=off, float_type=single, frac_width=0, exp_width=0}
      mask prompts: n_inputs "Number of Inputs"; latency "Add Latency"; adder_imp "Adder implementation"; first_stage_hdl "Use behavioural HDL for first stage of adders"; floating_point "floating point"; float_type "float type"; frac_width "fraction length"; exp_width "exponent length"
      mask help:
      | Sums all inputs using a tree of adds and delays.
      |
      | Number of inputs: The number of inputs to the block to be summed
      | Add latency: The number of clock cycles to perform one addition (affects timing)..
      | Adder implementation: choice of fabric or DSP48E core, or behavioral HDL
      | Use behavioural HDL for first stage of adders: Causes the first stage of adders to be absorbed into DSP blocks if multipliers precede them (Virtex 5). Overrides Adder implementation
      mask init: same as s_c_nbe_m32k/DDC/dec_fir_async/imag_sum
      settings: AttributesFormatString=latency 5
      mask Help: eval('xlWeb(''http://casper.berkeley.edu/wiki/Adder_tree'')')
      mask TypeOptions adder_imp: Behavioral | Fabric | DSP48
      mask Callback floating_point:
      | onoff = get_param(gcb, 'floating_point');
      | if strcmp(onoff,'on')
      |     enable_fixpt = 'off'
      |     set_param_state(gcb, 'float_type', 'on')
      | 
      |     f_type = get_param(gcb, 'float_type')
      |     if strcmp(f_type,'custom')
      |         set_param_state(gcb, 'exp_width', 'on')
      |         set_param_state(gcb, 'frac_width', 'on')
      |     else
      |         set_param_state(gcb, 'exp_width', 'off')
      |         set_param_state(gcb, 'frac_width', 'off')
      |     end
      | 
      | 
      | else
      |     enable_fixpt = 'on'
      |     set_param_state(gcb, 'float_type', 'off')
      |     set_param_state(gcb, 'exp_width', 'off')
      |     set_param_state(gcb, 'frac_width', 'off')
      | end
      mask TypeOptions float_type: single | custom
      mask Callback float_type:
      | f_type = get_param(gcb, 'float_type')
      | if strcmp(f_type,'custom')
      |     set_param_state(gcb, 'exp_width', 'on')
      |     set_param_state(gcb, 'frac_width', 'on')
      | else
      |     set_param_state(gcb, 'exp_width', 'off')
      |     set_param_state(gcb, 'frac_width', 'off')
      | end
  ri_to_c : casper_library_misc/ri_to_c
  shift1 : xbsIndex_r4/Shift  shift_dir=Left  shift_bits=1  en=off  latency=1  precision=Full  arith_type="Signed  (2's comp)"  n_bits=16  bin_pt=14  quantization=Truncate  overflow=Wrap  dbl_ovrd=off  block_type=shift
  shift2 : xbsIndex_r4/Shift  shift_dir=Left  shift_bits=1  en=off  latency=1  precision=Full  arith_type="Signed  (2's comp)"  n_bits=16  bin_pt=14  quantization=Truncate  overflow=Wrap  dbl_ovrd=off  block_type=shift
  sync_delay : xbsIndex_r4/Delay  rst=off  infoeditControl=Selection of Reset will increase slice count due to use of real FFs and instead of SRLs  en=off  latency=8  reg_retiming=off  dbl_ovrd=off  block_type=delay
      settings: infoedit=Hardware notes: A delay line is a chain, each link of which is an SRL16 or SRL32 followed by a flip-flop.
  sync_out : Outport
  dout : Outport  Port=2
  dv_out : Outport  Port=3
  wires:
  sync_in/1 -> sync_delay/1
  dv_in/1 -> dv_delay/1, fir_col_async1/33(dv), fir_col_async2/33(dv), fir_col_async3/33(dv), fir_col_async4/33(dv), fir_col_async5/33(dv), fir_col_async6/33(dv), fir_col_async7/33(dv), fir_col_async8/33(dv), fir_col_async9/33(dv), fir_col_async10/33(dv), fir_col_async11/33(dv), fir_col_async12/33(dv), fir_col_async13/33(dv), fir_col_async14/33(dv), fir_col_async15/33(dv), fir_col_async16/33(dv), fir_col_async17/33(dv), fir_col_async18/33(dv), fir_col_async19/33(dv), fir_col_async20/33(dv), fir_col_async21/33(dv), fir_col_async22/33(dv), fir_col_async23/33(dv), fir_col_async24/33(dv), fir_col_async25/33(dv), fir_col_async26/33(dv), fir_col_async27/33(dv), fir_col_async28/33(dv), fir_col_async29/33(dv), fir_col_async30/33(dv), fir_col_async31/33(dv), fir_col_async32/33(dv)
  dv_delay/1 -> dv_out/1
  real1/1 -> fir_col_async1/1(real1)
  imag1/1 -> fir_col_async1/2(imag1)
  real2/1 -> fir_col_async1/3(real2)
  imag2/1 -> fir_col_async1/4(imag2)
  real3/1 -> fir_col_async1/5(real3)
  imag3/1 -> fir_col_async1/6(imag3)
  real4/1 -> fir_col_async1/7(real4)
  imag4/1 -> fir_col_async1/8(imag4)
  real5/1 -> fir_col_async1/9(real5)
  imag5/1 -> fir_col_async1/10(imag5)
  real6/1 -> fir_col_async1/11(real6)
  imag6/1 -> fir_col_async1/12(imag6)
  real7/1 -> fir_col_async1/13(real7)
  imag7/1 -> fir_col_async1/14(imag7)
  real8/1 -> fir_col_async1/15(real8)
  imag8/1 -> fir_col_async1/16(imag8)
  fir_col_async1/33(real_sum) -> real_sum/2(din1)
  fir_col_async1/34(imag_sum) -> imag_sum/2(din1)
  fir_col_async1/1(real_out1) -> fir_col_async2/1(real1)
  fir_col_async1/2(imag_out1) -> fir_col_async2/2(imag1)
  fir_col_async1/3(real_out2) -> fir_col_async2/3(real2)
  fir_col_async1/4(imag_out2) -> fir_col_async2/4(imag2)
  fir_col_async1/5(real_out3) -> fir_col_async2/5(real3)
  fir_col_async1/6(imag_out3) -> fir_col_async2/6(imag3)
  fir_col_async1/7(real_out4) -> fir_col_async2/7(real4)
  fir_col_async1/8(imag_out4) -> fir_col_async2/8(imag4)
  fir_col_async1/9(real_out5) -> fir_col_async2/9(real5)
  fir_col_async1/10(imag_out5) -> fir_col_async2/10(imag5)
  fir_col_async1/11(real_out6) -> fir_col_async2/11(real6)
  fir_col_async1/12(imag_out6) -> fir_col_async2/12(imag6)
  fir_col_async1/13(real_out7) -> fir_col_async2/13(real7)
  fir_col_async1/14(imag_out7) -> fir_col_async2/14(imag7)
  fir_col_async1/15(real_out8) -> fir_col_async2/15(real8)
  fir_col_async1/16(imag_out8) -> fir_col_async2/16(imag8)
  fir_col_async2/33(real_sum) -> real_sum/3(din2)
  fir_col_async2/34(imag_sum) -> imag_sum/3(din2)
  fir_col_async2/1(real_out1) -> fir_col_async3/1(real1)
  fir_col_async2/2(imag_out1) -> fir_col_async3/2(imag1)
  fir_col_async2/3(real_out2) -> fir_col_async3/3(real2)
  fir_col_async2/4(imag_out2) -> fir_col_async3/4(imag2)
  fir_col_async2/5(real_out3) -> fir_col_async3/5(real3)
  fir_col_async2/6(imag_out3) -> fir_col_async3/6(imag3)
  fir_col_async2/7(real_out4) -> fir_col_async3/7(real4)
  fir_col_async2/8(imag_out4) -> fir_col_async3/8(imag4)
  fir_col_async2/9(real_out5) -> fir_col_async3/9(real5)
  fir_col_async2/10(imag_out5) -> fir_col_async3/10(imag5)
  fir_col_async2/11(real_out6) -> fir_col_async3/11(real6)
  fir_col_async2/12(imag_out6) -> fir_col_async3/12(imag6)
  fir_col_async2/13(real_out7) -> fir_col_async3/13(real7)
  fir_col_async2/14(imag_out7) -> fir_col_async3/14(imag7)
  fir_col_async2/15(real_out8) -> fir_col_async3/15(real8)
  fir_col_async2/16(imag_out8) -> fir_col_async3/16(imag8)
  fir_col_async3/33(real_sum) -> real_sum/4(din3)
  fir_col_async3/34(imag_sum) -> imag_sum/4(din3)
  fir_col_async3/1(real_out1) -> fir_col_async4/1(real1)
  fir_col_async3/2(imag_out1) -> fir_col_async4/2(imag1)
  fir_col_async3/3(real_out2) -> fir_col_async4/3(real2)
  fir_col_async3/4(imag_out2) -> fir_col_async4/4(imag2)
  fir_col_async3/5(real_out3) -> fir_col_async4/5(real3)
  fir_col_async3/6(imag_out3) -> fir_col_async4/6(imag3)
  fir_col_async3/7(real_out4) -> fir_col_async4/7(real4)
  fir_col_async3/8(imag_out4) -> fir_col_async4/8(imag4)
  fir_col_async3/9(real_out5) -> fir_col_async4/9(real5)
  fir_col_async3/10(imag_out5) -> fir_col_async4/10(imag5)
  fir_col_async3/11(real_out6) -> fir_col_async4/11(real6)
  fir_col_async3/12(imag_out6) -> fir_col_async4/12(imag6)
  fir_col_async3/13(real_out7) -> fir_col_async4/13(real7)
  fir_col_async3/14(imag_out7) -> fir_col_async4/14(imag7)
  fir_col_async3/15(real_out8) -> fir_col_async4/15(real8)
  fir_col_async3/16(imag_out8) -> fir_col_async4/16(imag8)
  fir_col_async4/33(real_sum) -> real_sum/5(din4)
  fir_col_async4/34(imag_sum) -> imag_sum/5(din4)
  fir_col_async4/1(real_out1) -> fir_col_async5/1(real1)
  fir_col_async4/2(imag_out1) -> fir_col_async5/2(imag1)
  fir_col_async4/3(real_out2) -> fir_col_async5/3(real2)
  fir_col_async4/4(imag_out2) -> fir_col_async5/4(imag2)
  fir_col_async4/5(real_out3) -> fir_col_async5/5(real3)
  fir_col_async4/6(imag_out3) -> fir_col_async5/6(imag3)
  fir_col_async4/7(real_out4) -> fir_col_async5/7(real4)
  fir_col_async4/8(imag_out4) -> fir_col_async5/8(imag4)
  fir_col_async4/9(real_out5) -> fir_col_async5/9(real5)
  fir_col_async4/10(imag_out5) -> fir_col_async5/10(imag5)
  fir_col_async4/11(real_out6) -> fir_col_async5/11(real6)
  fir_col_async4/12(imag_out6) -> fir_col_async5/12(imag6)
  fir_col_async4/13(real_out7) -> fir_col_async5/13(real7)
  fir_col_async4/14(imag_out7) -> fir_col_async5/14(imag7)
  fir_col_async4/15(real_out8) -> fir_col_async5/15(real8)
  fir_col_async4/16(imag_out8) -> fir_col_async5/16(imag8)
  fir_col_async5/33(real_sum) -> real_sum/6(din5)
  fir_col_async5/34(imag_sum) -> imag_sum/6(din5)
  fir_col_async5/1(real_out1) -> fir_col_async6/1(real1)
  fir_col_async5/2(imag_out1) -> fir_col_async6/2(imag1)
  fir_col_async5/3(real_out2) -> fir_col_async6/3(real2)
  fir_col_async5/4(imag_out2) -> fir_col_async6/4(imag2)
  fir_col_async5/5(real_out3) -> fir_col_async6/5(real3)
  fir_col_async5/6(imag_out3) -> fir_col_async6/6(imag3)
  fir_col_async5/7(real_out4) -> fir_col_async6/7(real4)
  fir_col_async5/8(imag_out4) -> fir_col_async6/8(imag4)
  fir_col_async5/9(real_out5) -> fir_col_async6/9(real5)
  fir_col_async5/10(imag_out5) -> fir_col_async6/10(imag5)
  fir_col_async5/11(real_out6) -> fir_col_async6/11(real6)
  fir_col_async5/12(imag_out6) -> fir_col_async6/12(imag6)
  fir_col_async5/13(real_out7) -> fir_col_async6/13(real7)
  fir_col_async5/14(imag_out7) -> fir_col_async6/14(imag7)
  fir_col_async5/15(real_out8) -> fir_col_async6/15(real8)
  fir_col_async5/16(imag_out8) -> fir_col_async6/16(imag8)
  fir_col_async6/33(real_sum) -> real_sum/7(din6)
  fir_col_async6/34(imag_sum) -> imag_sum/7(din6)
  fir_col_async6/1(real_out1) -> fir_col_async7/1(real1)
  fir_col_async6/2(imag_out1) -> fir_col_async7/2(imag1)
  fir_col_async6/3(real_out2) -> fir_col_async7/3(real2)
  fir_col_async6/4(imag_out2) -> fir_col_async7/4(imag2)
  fir_col_async6/5(real_out3) -> fir_col_async7/5(real3)
  fir_col_async6/6(imag_out3) -> fir_col_async7/6(imag3)
  fir_col_async6/7(real_out4) -> fir_col_async7/7(real4)
  fir_col_async6/8(imag_out4) -> fir_col_async7/8(imag4)
  fir_col_async6/9(real_out5) -> fir_col_async7/9(real5)
  fir_col_async6/10(imag_out5) -> fir_col_async7/10(imag5)
  fir_col_async6/11(real_out6) -> fir_col_async7/11(real6)
  fir_col_async6/12(imag_out6) -> fir_col_async7/12(imag6)
  fir_col_async6/13(real_out7) -> fir_col_async7/13(real7)
  fir_col_async6/14(imag_out7) -> fir_col_async7/14(imag7)
  fir_col_async6/15(real_out8) -> fir_col_async7/15(real8)
  fir_col_async6/16(imag_out8) -> fir_col_async7/16(imag8)
  fir_col_async7/33(real_sum) -> real_sum/8(din7)
  fir_col_async7/34(imag_sum) -> imag_sum/8(din7)
  fir_col_async7/1(real_out1) -> fir_col_async8/1(real1)
  fir_col_async7/2(imag_out1) -> fir_col_async8/2(imag1)
  fir_col_async7/3(real_out2) -> fir_col_async8/3(real2)
  fir_col_async7/4(imag_out2) -> fir_col_async8/4(imag2)
  fir_col_async7/5(real_out3) -> fir_col_async8/5(real3)
  fir_col_async7/6(imag_out3) -> fir_col_async8/6(imag3)
  fir_col_async7/7(real_out4) -> fir_col_async8/7(real4)
  fir_col_async7/8(imag_out4) -> fir_col_async8/8(imag4)
  fir_col_async7/9(real_out5) -> fir_col_async8/9(real5)
  fir_col_async7/10(imag_out5) -> fir_col_async8/10(imag5)
  fir_col_async7/11(real_out6) -> fir_col_async8/11(real6)
  fir_col_async7/12(imag_out6) -> fir_col_async8/12(imag6)
  fir_col_async7/13(real_out7) -> fir_col_async8/13(real7)
  fir_col_async7/14(imag_out7) -> fir_col_async8/14(imag7)
  fir_col_async7/15(real_out8) -> fir_col_async8/15(real8)
  fir_col_async7/16(imag_out8) -> fir_col_async8/16(imag8)
  fir_col_async8/33(real_sum) -> real_sum/9(din8)
  fir_col_async8/34(imag_sum) -> imag_sum/9(din8)
  fir_col_async8/1(real_out1) -> fir_col_async9/1(real1)
  fir_col_async8/2(imag_out1) -> fir_col_async9/2(imag1)
  fir_col_async8/3(real_out2) -> fir_col_async9/3(real2)
  fir_col_async8/4(imag_out2) -> fir_col_async9/4(imag2)
  fir_col_async8/5(real_out3) -> fir_col_async9/5(real3)
  fir_col_async8/6(imag_out3) -> fir_col_async9/6(imag3)
  fir_col_async8/7(real_out4) -> fir_col_async9/7(real4)
  fir_col_async8/8(imag_out4) -> fir_col_async9/8(imag4)
  fir_col_async8/9(real_out5) -> fir_col_async9/9(real5)
  fir_col_async8/10(imag_out5) -> fir_col_async9/10(imag5)
  fir_col_async8/11(real_out6) -> fir_col_async9/11(real6)
  fir_col_async8/12(imag_out6) -> fir_col_async9/12(imag6)
  fir_col_async8/13(real_out7) -> fir_col_async9/13(real7)
  fir_col_async8/14(imag_out7) -> fir_col_async9/14(imag7)
  fir_col_async8/15(real_out8) -> fir_col_async9/15(real8)
  fir_col_async8/16(imag_out8) -> fir_col_async9/16(imag8)
  fir_col_async9/33(real_sum) -> real_sum/10(din9)
  fir_col_async9/34(imag_sum) -> imag_sum/10(din9)
  fir_col_async9/1(real_out1) -> fir_col_async10/1(real1)
  fir_col_async9/2(imag_out1) -> fir_col_async10/2(imag1)
  fir_col_async9/3(real_out2) -> fir_col_async10/3(real2)
  fir_col_async9/4(imag_out2) -> fir_col_async10/4(imag2)
  fir_col_async9/5(real_out3) -> fir_col_async10/5(real3)
  fir_col_async9/6(imag_out3) -> fir_col_async10/6(imag3)
  fir_col_async9/7(real_out4) -> fir_col_async10/7(real4)
  fir_col_async9/8(imag_out4) -> fir_col_async10/8(imag4)
  fir_col_async9/9(real_out5) -> fir_col_async10/9(real5)
  fir_col_async9/10(imag_out5) -> fir_col_async10/10(imag5)
  fir_col_async9/11(real_out6) -> fir_col_async10/11(real6)
  fir_col_async9/12(imag_out6) -> fir_col_async10/12(imag6)
  fir_col_async9/13(real_out7) -> fir_col_async10/13(real7)
  fir_col_async9/14(imag_out7) -> fir_col_async10/14(imag7)
  fir_col_async9/15(real_out8) -> fir_col_async10/15(real8)
  fir_col_async9/16(imag_out8) -> fir_col_async10/16(imag8)
  fir_col_async10/33(real_sum) -> real_sum/11(din10)
  fir_col_async10/34(imag_sum) -> imag_sum/11(din10)
  fir_col_async10/1(real_out1) -> fir_col_async11/1(real1)
  fir_col_async10/2(imag_out1) -> fir_col_async11/2(imag1)
  fir_col_async10/3(real_out2) -> fir_col_async11/3(real2)
  fir_col_async10/4(imag_out2) -> fir_col_async11/4(imag2)
  fir_col_async10/5(real_out3) -> fir_col_async11/5(real3)
  fir_col_async10/6(imag_out3) -> fir_col_async11/6(imag3)
  fir_col_async10/7(real_out4) -> fir_col_async11/7(real4)
  fir_col_async10/8(imag_out4) -> fir_col_async11/8(imag4)
  fir_col_async10/9(real_out5) -> fir_col_async11/9(real5)
  fir_col_async10/10(imag_out5) -> fir_col_async11/10(imag5)
  fir_col_async10/11(real_out6) -> fir_col_async11/11(real6)
  fir_col_async10/12(imag_out6) -> fir_col_async11/12(imag6)
  fir_col_async10/13(real_out7) -> fir_col_async11/13(real7)
  fir_col_async10/14(imag_out7) -> fir_col_async11/14(imag7)
  fir_col_async10/15(real_out8) -> fir_col_async11/15(real8)
  fir_col_async10/16(imag_out8) -> fir_col_async11/16(imag8)
  fir_col_async11/33(real_sum) -> real_sum/12(din11)
  fir_col_async11/34(imag_sum) -> imag_sum/12(din11)
  fir_col_async11/1(real_out1) -> fir_col_async12/1(real1)
  fir_col_async11/2(imag_out1) -> fir_col_async12/2(imag1)
  fir_col_async11/3(real_out2) -> fir_col_async12/3(real2)
  fir_col_async11/4(imag_out2) -> fir_col_async12/4(imag2)
  fir_col_async11/5(real_out3) -> fir_col_async12/5(real3)
  fir_col_async11/6(imag_out3) -> fir_col_async12/6(imag3)
  fir_col_async11/7(real_out4) -> fir_col_async12/7(real4)
  fir_col_async11/8(imag_out4) -> fir_col_async12/8(imag4)
  fir_col_async11/9(real_out5) -> fir_col_async12/9(real5)
  fir_col_async11/10(imag_out5) -> fir_col_async12/10(imag5)
  fir_col_async11/11(real_out6) -> fir_col_async12/11(real6)
  fir_col_async11/12(imag_out6) -> fir_col_async12/12(imag6)
  fir_col_async11/13(real_out7) -> fir_col_async12/13(real7)
  fir_col_async11/14(imag_out7) -> fir_col_async12/14(imag7)
  fir_col_async11/15(real_out8) -> fir_col_async12/15(real8)
  fir_col_async11/16(imag_out8) -> fir_col_async12/16(imag8)
  fir_col_async12/33(real_sum) -> real_sum/13(din12)
  fir_col_async12/34(imag_sum) -> imag_sum/13(din12)
  fir_col_async12/1(real_out1) -> fir_col_async13/1(real1)
  fir_col_async12/2(imag_out1) -> fir_col_async13/2(imag1)
  fir_col_async12/3(real_out2) -> fir_col_async13/3(real2)
  fir_col_async12/4(imag_out2) -> fir_col_async13/4(imag2)
  fir_col_async12/5(real_out3) -> fir_col_async13/5(real3)
  fir_col_async12/6(imag_out3) -> fir_col_async13/6(imag3)
  fir_col_async12/7(real_out4) -> fir_col_async13/7(real4)
  fir_col_async12/8(imag_out4) -> fir_col_async13/8(imag4)
  fir_col_async12/9(real_out5) -> fir_col_async13/9(real5)
  fir_col_async12/10(imag_out5) -> fir_col_async13/10(imag5)
  fir_col_async12/11(real_out6) -> fir_col_async13/11(real6)
  fir_col_async12/12(imag_out6) -> fir_col_async13/12(imag6)
  fir_col_async12/13(real_out7) -> fir_col_async13/13(real7)
  fir_col_async12/14(imag_out7) -> fir_col_async13/14(imag7)
  fir_col_async12/15(real_out8) -> fir_col_async13/15(real8)
  fir_col_async12/16(imag_out8) -> fir_col_async13/16(imag8)
  fir_col_async13/33(real_sum) -> real_sum/14(din13)
  fir_col_async13/34(imag_sum) -> imag_sum/14(din13)
  fir_col_async13/1(real_out1) -> fir_col_async14/1(real1)
  fir_col_async13/2(imag_out1) -> fir_col_async14/2(imag1)
  fir_col_async13/3(real_out2) -> fir_col_async14/3(real2)
  fir_col_async13/4(imag_out2) -> fir_col_async14/4(imag2)
  fir_col_async13/5(real_out3) -> fir_col_async14/5(real3)
  fir_col_async13/6(imag_out3) -> fir_col_async14/6(imag3)
  fir_col_async13/7(real_out4) -> fir_col_async14/7(real4)
  fir_col_async13/8(imag_out4) -> fir_col_async14/8(imag4)
  fir_col_async13/9(real_out5) -> fir_col_async14/9(real5)
  fir_col_async13/10(imag_out5) -> fir_col_async14/10(imag5)
  fir_col_async13/11(real_out6) -> fir_col_async14/11(real6)
  fir_col_async13/12(imag_out6) -> fir_col_async14/12(imag6)
  fir_col_async13/13(real_out7) -> fir_col_async14/13(real7)
  fir_col_async13/14(imag_out7) -> fir_col_async14/14(imag7)
  fir_col_async13/15(real_out8) -> fir_col_async14/15(real8)
  fir_col_async13/16(imag_out8) -> fir_col_async14/16(imag8)
  fir_col_async14/33(real_sum) -> real_sum/15(din14)
  fir_col_async14/34(imag_sum) -> imag_sum/15(din14)
  fir_col_async14/1(real_out1) -> fir_col_async15/1(real1)
  fir_col_async14/2(imag_out1) -> fir_col_async15/2(imag1)
  fir_col_async14/3(real_out2) -> fir_col_async15/3(real2)
  fir_col_async14/4(imag_out2) -> fir_col_async15/4(imag2)
  fir_col_async14/5(real_out3) -> fir_col_async15/5(real3)
  fir_col_async14/6(imag_out3) -> fir_col_async15/6(imag3)
  fir_col_async14/7(real_out4) -> fir_col_async15/7(real4)
  fir_col_async14/8(imag_out4) -> fir_col_async15/8(imag4)
  fir_col_async14/9(real_out5) -> fir_col_async15/9(real5)
  fir_col_async14/10(imag_out5) -> fir_col_async15/10(imag5)
  fir_col_async14/11(real_out6) -> fir_col_async15/11(real6)
  fir_col_async14/12(imag_out6) -> fir_col_async15/12(imag6)
  fir_col_async14/13(real_out7) -> fir_col_async15/13(real7)
  fir_col_async14/14(imag_out7) -> fir_col_async15/14(imag7)
  fir_col_async14/15(real_out8) -> fir_col_async15/15(real8)
  fir_col_async14/16(imag_out8) -> fir_col_async15/16(imag8)
  fir_col_async15/33(real_sum) -> real_sum/16(din15)
  fir_col_async15/34(imag_sum) -> imag_sum/16(din15)
  fir_col_async15/1(real_out1) -> fir_col_async16/1(real1)
  fir_col_async15/2(imag_out1) -> fir_col_async16/2(imag1)
  fir_col_async15/3(real_out2) -> fir_col_async16/3(real2)
  fir_col_async15/4(imag_out2) -> fir_col_async16/4(imag2)
  fir_col_async15/5(real_out3) -> fir_col_async16/5(real3)
  fir_col_async15/6(imag_out3) -> fir_col_async16/6(imag3)
  fir_col_async15/7(real_out4) -> fir_col_async16/7(real4)
  fir_col_async15/8(imag_out4) -> fir_col_async16/8(imag4)
  fir_col_async15/9(real_out5) -> fir_col_async16/9(real5)
  fir_col_async15/10(imag_out5) -> fir_col_async16/10(imag5)
  fir_col_async15/11(real_out6) -> fir_col_async16/11(real6)
  fir_col_async15/12(imag_out6) -> fir_col_async16/12(imag6)
  fir_col_async15/13(real_out7) -> fir_col_async16/13(real7)
  fir_col_async15/14(imag_out7) -> fir_col_async16/14(imag7)
  fir_col_async15/15(real_out8) -> fir_col_async16/15(real8)
  fir_col_async15/16(imag_out8) -> fir_col_async16/16(imag8)
  fir_col_async16/33(real_sum) -> real_sum/17(din16)
  fir_col_async16/34(imag_sum) -> imag_sum/17(din16)
  fir_col_async16/1(real_out1) -> fir_col_async17/1(real1)
  fir_col_async16/2(imag_out1) -> fir_col_async17/2(imag1)
  fir_col_async16/3(real_out2) -> fir_col_async17/3(real2)
  fir_col_async16/4(imag_out2) -> fir_col_async17/4(imag2)
  fir_col_async16/5(real_out3) -> fir_col_async17/5(real3)
  fir_col_async16/6(imag_out3) -> fir_col_async17/6(imag3)
  fir_col_async16/7(real_out4) -> fir_col_async17/7(real4)
  fir_col_async16/8(imag_out4) -> fir_col_async17/8(imag4)
  fir_col_async16/9(real_out5) -> fir_col_async17/9(real5)
  fir_col_async16/10(imag_out5) -> fir_col_async17/10(imag5)
  fir_col_async16/11(real_out6) -> fir_col_async17/11(real6)
  fir_col_async16/12(imag_out6) -> fir_col_async17/12(imag6)
  fir_col_async16/13(real_out7) -> fir_col_async17/13(real7)
  fir_col_async16/14(imag_out7) -> fir_col_async17/14(imag7)
  fir_col_async16/15(real_out8) -> fir_col_async17/15(real8)
  fir_col_async16/16(imag_out8) -> fir_col_async17/16(imag8)
  fir_col_async17/33(real_sum) -> real_sum/18(din17)
  fir_col_async17/34(imag_sum) -> imag_sum/18(din17)
  fir_col_async17/1(real_out1) -> fir_col_async18/1(real1)
  fir_col_async17/2(imag_out1) -> fir_col_async18/2(imag1)
  fir_col_async17/3(real_out2) -> fir_col_async18/3(real2)
  fir_col_async17/4(imag_out2) -> fir_col_async18/4(imag2)
  fir_col_async17/5(real_out3) -> fir_col_async18/5(real3)
  fir_col_async17/6(imag_out3) -> fir_col_async18/6(imag3)
  fir_col_async17/7(real_out4) -> fir_col_async18/7(real4)
  fir_col_async17/8(imag_out4) -> fir_col_async18/8(imag4)
  fir_col_async17/9(real_out5) -> fir_col_async18/9(real5)
  fir_col_async17/10(imag_out5) -> fir_col_async18/10(imag5)
  fir_col_async17/11(real_out6) -> fir_col_async18/11(real6)
  fir_col_async17/12(imag_out6) -> fir_col_async18/12(imag6)
  fir_col_async17/13(real_out7) -> fir_col_async18/13(real7)
  fir_col_async17/14(imag_out7) -> fir_col_async18/14(imag7)
  fir_col_async17/15(real_out8) -> fir_col_async18/15(real8)
  fir_col_async17/16(imag_out8) -> fir_col_async18/16(imag8)
  fir_col_async18/33(real_sum) -> real_sum/19(din18)
  fir_col_async18/34(imag_sum) -> imag_sum/19(din18)
  fir_col_async18/1(real_out1) -> fir_col_async19/1(real1)
  fir_col_async18/2(imag_out1) -> fir_col_async19/2(imag1)
  fir_col_async18/3(real_out2) -> fir_col_async19/3(real2)
  fir_col_async18/4(imag_out2) -> fir_col_async19/4(imag2)
  fir_col_async18/5(real_out3) -> fir_col_async19/5(real3)
  fir_col_async18/6(imag_out3) -> fir_col_async19/6(imag3)
  fir_col_async18/7(real_out4) -> fir_col_async19/7(real4)
  fir_col_async18/8(imag_out4) -> fir_col_async19/8(imag4)
  fir_col_async18/9(real_out5) -> fir_col_async19/9(real5)
  fir_col_async18/10(imag_out5) -> fir_col_async19/10(imag5)
  fir_col_async18/11(real_out6) -> fir_col_async19/11(real6)
  fir_col_async18/12(imag_out6) -> fir_col_async19/12(imag6)
  fir_col_async18/13(real_out7) -> fir_col_async19/13(real7)
  fir_col_async18/14(imag_out7) -> fir_col_async19/14(imag7)
  fir_col_async18/15(real_out8) -> fir_col_async19/15(real8)
  fir_col_async18/16(imag_out8) -> fir_col_async19/16(imag8)
  fir_col_async19/33(real_sum) -> real_sum/20(din19)
  fir_col_async19/34(imag_sum) -> imag_sum/20(din19)
  fir_col_async19/1(real_out1) -> fir_col_async20/1(real1)
  fir_col_async19/2(imag_out1) -> fir_col_async20/2(imag1)
  fir_col_async19/3(real_out2) -> fir_col_async20/3(real2)
  fir_col_async19/4(imag_out2) -> fir_col_async20/4(imag2)
  fir_col_async19/5(real_out3) -> fir_col_async20/5(real3)
  fir_col_async19/6(imag_out3) -> fir_col_async20/6(imag3)
  fir_col_async19/7(real_out4) -> fir_col_async20/7(real4)
  fir_col_async19/8(imag_out4) -> fir_col_async20/8(imag4)
  fir_col_async19/9(real_out5) -> fir_col_async20/9(real5)
  fir_col_async19/10(imag_out5) -> fir_col_async20/10(imag5)
  fir_col_async19/11(real_out6) -> fir_col_async20/11(real6)
  fir_col_async19/12(imag_out6) -> fir_col_async20/12(imag6)
  fir_col_async19/13(real_out7) -> fir_col_async20/13(real7)
  fir_col_async19/14(imag_out7) -> fir_col_async20/14(imag7)
  fir_col_async19/15(real_out8) -> fir_col_async20/15(real8)
  fir_col_async19/16(imag_out8) -> fir_col_async20/16(imag8)
  fir_col_async20/33(real_sum) -> real_sum/21(din20)
  fir_col_async20/34(imag_sum) -> imag_sum/21(din20)
  fir_col_async20/1(real_out1) -> fir_col_async21/1(real1)
  fir_col_async20/2(imag_out1) -> fir_col_async21/2(imag1)
  fir_col_async20/3(real_out2) -> fir_col_async21/3(real2)
  fir_col_async20/4(imag_out2) -> fir_col_async21/4(imag2)
  fir_col_async20/5(real_out3) -> fir_col_async21/5(real3)
  fir_col_async20/6(imag_out3) -> fir_col_async21/6(imag3)
  fir_col_async20/7(real_out4) -> fir_col_async21/7(real4)
  fir_col_async20/8(imag_out4) -> fir_col_async21/8(imag4)
  fir_col_async20/9(real_out5) -> fir_col_async21/9(real5)
  fir_col_async20/10(imag_out5) -> fir_col_async21/10(imag5)
  fir_col_async20/11(real_out6) -> fir_col_async21/11(real6)
  fir_col_async20/12(imag_out6) -> fir_col_async21/12(imag6)
  fir_col_async20/13(real_out7) -> fir_col_async21/13(real7)
  fir_col_async20/14(imag_out7) -> fir_col_async21/14(imag7)
  fir_col_async20/15(real_out8) -> fir_col_async21/15(real8)
  fir_col_async20/16(imag_out8) -> fir_col_async21/16(imag8)
  fir_col_async21/33(real_sum) -> real_sum/22(din21)
  fir_col_async21/34(imag_sum) -> imag_sum/22(din21)
  fir_col_async21/1(real_out1) -> fir_col_async22/1(real1)
  fir_col_async21/2(imag_out1) -> fir_col_async22/2(imag1)
  fir_col_async21/3(real_out2) -> fir_col_async22/3(real2)
  fir_col_async21/4(imag_out2) -> fir_col_async22/4(imag2)
  fir_col_async21/5(real_out3) -> fir_col_async22/5(real3)
  fir_col_async21/6(imag_out3) -> fir_col_async22/6(imag3)
  fir_col_async21/7(real_out4) -> fir_col_async22/7(real4)
  fir_col_async21/8(imag_out4) -> fir_col_async22/8(imag4)
  fir_col_async21/9(real_out5) -> fir_col_async22/9(real5)
  fir_col_async21/10(imag_out5) -> fir_col_async22/10(imag5)
  fir_col_async21/11(real_out6) -> fir_col_async22/11(real6)
  fir_col_async21/12(imag_out6) -> fir_col_async22/12(imag6)
  fir_col_async21/13(real_out7) -> fir_col_async22/13(real7)
  fir_col_async21/14(imag_out7) -> fir_col_async22/14(imag7)
  fir_col_async21/15(real_out8) -> fir_col_async22/15(real8)
  fir_col_async21/16(imag_out8) -> fir_col_async22/16(imag8)
  fir_col_async22/33(real_sum) -> real_sum/23(din22)
  fir_col_async22/34(imag_sum) -> imag_sum/23(din22)
  fir_col_async22/1(real_out1) -> fir_col_async23/1(real1)
  fir_col_async22/2(imag_out1) -> fir_col_async23/2(imag1)
  fir_col_async22/3(real_out2) -> fir_col_async23/3(real2)
  fir_col_async22/4(imag_out2) -> fir_col_async23/4(imag2)
  fir_col_async22/5(real_out3) -> fir_col_async23/5(real3)
  fir_col_async22/6(imag_out3) -> fir_col_async23/6(imag3)
  fir_col_async22/7(real_out4) -> fir_col_async23/7(real4)
  fir_col_async22/8(imag_out4) -> fir_col_async23/8(imag4)
  fir_col_async22/9(real_out5) -> fir_col_async23/9(real5)
  fir_col_async22/10(imag_out5) -> fir_col_async23/10(imag5)
  fir_col_async22/11(real_out6) -> fir_col_async23/11(real6)
  fir_col_async22/12(imag_out6) -> fir_col_async23/12(imag6)
  fir_col_async22/13(real_out7) -> fir_col_async23/13(real7)
  fir_col_async22/14(imag_out7) -> fir_col_async23/14(imag7)
  fir_col_async22/15(real_out8) -> fir_col_async23/15(real8)
  fir_col_async22/16(imag_out8) -> fir_col_async23/16(imag8)
  fir_col_async23/33(real_sum) -> real_sum/24(din23)
  fir_col_async23/34(imag_sum) -> imag_sum/24(din23)
  fir_col_async23/1(real_out1) -> fir_col_async24/1(real1)
  fir_col_async23/2(imag_out1) -> fir_col_async24/2(imag1)
  fir_col_async23/3(real_out2) -> fir_col_async24/3(real2)
  fir_col_async23/4(imag_out2) -> fir_col_async24/4(imag2)
  fir_col_async23/5(real_out3) -> fir_col_async24/5(real3)
  fir_col_async23/6(imag_out3) -> fir_col_async24/6(imag3)
  fir_col_async23/7(real_out4) -> fir_col_async24/7(real4)
  fir_col_async23/8(imag_out4) -> fir_col_async24/8(imag4)
  fir_col_async23/9(real_out5) -> fir_col_async24/9(real5)
  fir_col_async23/10(imag_out5) -> fir_col_async24/10(imag5)
  fir_col_async23/11(real_out6) -> fir_col_async24/11(real6)
  fir_col_async23/12(imag_out6) -> fir_col_async24/12(imag6)
  fir_col_async23/13(real_out7) -> fir_col_async24/13(real7)
  fir_col_async23/14(imag_out7) -> fir_col_async24/14(imag7)
  fir_col_async23/15(real_out8) -> fir_col_async24/15(real8)
  fir_col_async23/16(imag_out8) -> fir_col_async24/16(imag8)
  fir_col_async24/33(real_sum) -> real_sum/25(din24)
  fir_col_async24/34(imag_sum) -> imag_sum/25(din24)
  fir_col_async24/1(real_out1) -> fir_col_async25/1(real1)
  fir_col_async24/2(imag_out1) -> fir_col_async25/2(imag1)
  fir_col_async24/3(real_out2) -> fir_col_async25/3(real2)
  fir_col_async24/4(imag_out2) -> fir_col_async25/4(imag2)
  fir_col_async24/5(real_out3) -> fir_col_async25/5(real3)
  fir_col_async24/6(imag_out3) -> fir_col_async25/6(imag3)
  fir_col_async24/7(real_out4) -> fir_col_async25/7(real4)
  fir_col_async24/8(imag_out4) -> fir_col_async25/8(imag4)
  fir_col_async24/9(real_out5) -> fir_col_async25/9(real5)
  fir_col_async24/10(imag_out5) -> fir_col_async25/10(imag5)
  fir_col_async24/11(real_out6) -> fir_col_async25/11(real6)
  fir_col_async24/12(imag_out6) -> fir_col_async25/12(imag6)
  fir_col_async24/13(real_out7) -> fir_col_async25/13(real7)
  fir_col_async24/14(imag_out7) -> fir_col_async25/14(imag7)
  fir_col_async24/15(real_out8) -> fir_col_async25/15(real8)
  fir_col_async24/16(imag_out8) -> fir_col_async25/16(imag8)
  fir_col_async25/33(real_sum) -> real_sum/26(din25)
  fir_col_async25/34(imag_sum) -> imag_sum/26(din25)
  fir_col_async25/1(real_out1) -> fir_col_async26/1(real1)
  fir_col_async25/2(imag_out1) -> fir_col_async26/2(imag1)
  fir_col_async25/3(real_out2) -> fir_col_async26/3(real2)
  fir_col_async25/4(imag_out2) -> fir_col_async26/4(imag2)
  fir_col_async25/5(real_out3) -> fir_col_async26/5(real3)
  fir_col_async25/6(imag_out3) -> fir_col_async26/6(imag3)
  fir_col_async25/7(real_out4) -> fir_col_async26/7(real4)
  fir_col_async25/8(imag_out4) -> fir_col_async26/8(imag4)
  fir_col_async25/9(real_out5) -> fir_col_async26/9(real5)
  fir_col_async25/10(imag_out5) -> fir_col_async26/10(imag5)
  fir_col_async25/11(real_out6) -> fir_col_async26/11(real6)
  fir_col_async25/12(imag_out6) -> fir_col_async26/12(imag6)
  fir_col_async25/13(real_out7) -> fir_col_async26/13(real7)
  fir_col_async25/14(imag_out7) -> fir_col_async26/14(imag7)
  fir_col_async25/15(real_out8) -> fir_col_async26/15(real8)
  fir_col_async25/16(imag_out8) -> fir_col_async26/16(imag8)
  fir_col_async26/33(real_sum) -> real_sum/27(din26)
  fir_col_async26/34(imag_sum) -> imag_sum/27(din26)
  fir_col_async26/1(real_out1) -> fir_col_async27/1(real1)
  fir_col_async26/2(imag_out1) -> fir_col_async27/2(imag1)
  fir_col_async26/3(real_out2) -> fir_col_async27/3(real2)
  fir_col_async26/4(imag_out2) -> fir_col_async27/4(imag2)
  fir_col_async26/5(real_out3) -> fir_col_async27/5(real3)
  fir_col_async26/6(imag_out3) -> fir_col_async27/6(imag3)
  fir_col_async26/7(real_out4) -> fir_col_async27/7(real4)
  fir_col_async26/8(imag_out4) -> fir_col_async27/8(imag4)
  fir_col_async26/9(real_out5) -> fir_col_async27/9(real5)
  fir_col_async26/10(imag_out5) -> fir_col_async27/10(imag5)
  fir_col_async26/11(real_out6) -> fir_col_async27/11(real6)
  fir_col_async26/12(imag_out6) -> fir_col_async27/12(imag6)
  fir_col_async26/13(real_out7) -> fir_col_async27/13(real7)
  fir_col_async26/14(imag_out7) -> fir_col_async27/14(imag7)
  fir_col_async26/15(real_out8) -> fir_col_async27/15(real8)
  fir_col_async26/16(imag_out8) -> fir_col_async27/16(imag8)
  fir_col_async27/33(real_sum) -> real_sum/28(din27)
  fir_col_async27/34(imag_sum) -> imag_sum/28(din27)
  fir_col_async27/1(real_out1) -> fir_col_async28/1(real1)
  fir_col_async27/2(imag_out1) -> fir_col_async28/2(imag1)
  fir_col_async27/3(real_out2) -> fir_col_async28/3(real2)
  fir_col_async27/4(imag_out2) -> fir_col_async28/4(imag2)
  fir_col_async27/5(real_out3) -> fir_col_async28/5(real3)
  fir_col_async27/6(imag_out3) -> fir_col_async28/6(imag3)
  fir_col_async27/7(real_out4) -> fir_col_async28/7(real4)
  fir_col_async27/8(imag_out4) -> fir_col_async28/8(imag4)
  fir_col_async27/9(real_out5) -> fir_col_async28/9(real5)
  fir_col_async27/10(imag_out5) -> fir_col_async28/10(imag5)
  fir_col_async27/11(real_out6) -> fir_col_async28/11(real6)
  fir_col_async27/12(imag_out6) -> fir_col_async28/12(imag6)
  fir_col_async27/13(real_out7) -> fir_col_async28/13(real7)
  fir_col_async27/14(imag_out7) -> fir_col_async28/14(imag7)
  fir_col_async27/15(real_out8) -> fir_col_async28/15(real8)
  fir_col_async27/16(imag_out8) -> fir_col_async28/16(imag8)
  fir_col_async28/33(real_sum) -> real_sum/29(din28)
  fir_col_async28/34(imag_sum) -> imag_sum/29(din28)
  fir_col_async28/1(real_out1) -> fir_col_async29/1(real1)
  fir_col_async28/2(imag_out1) -> fir_col_async29/2(imag1)
  fir_col_async28/3(real_out2) -> fir_col_async29/3(real2)
  fir_col_async28/4(imag_out2) -> fir_col_async29/4(imag2)
  fir_col_async28/5(real_out3) -> fir_col_async29/5(real3)
  fir_col_async28/6(imag_out3) -> fir_col_async29/6(imag3)
  fir_col_async28/7(real_out4) -> fir_col_async29/7(real4)
  fir_col_async28/8(imag_out4) -> fir_col_async29/8(imag4)
  fir_col_async28/9(real_out5) -> fir_col_async29/9(real5)
  fir_col_async28/10(imag_out5) -> fir_col_async29/10(imag5)
  fir_col_async28/11(real_out6) -> fir_col_async29/11(real6)
  fir_col_async28/12(imag_out6) -> fir_col_async29/12(imag6)
  fir_col_async28/13(real_out7) -> fir_col_async29/13(real7)
  fir_col_async28/14(imag_out7) -> fir_col_async29/14(imag7)
  fir_col_async28/15(real_out8) -> fir_col_async29/15(real8)
  fir_col_async28/16(imag_out8) -> fir_col_async29/16(imag8)
  fir_col_async29/33(real_sum) -> real_sum/30(din29)
  fir_col_async29/34(imag_sum) -> imag_sum/30(din29)
  fir_col_async29/1(real_out1) -> fir_col_async30/1(real1)
  fir_col_async29/2(imag_out1) -> fir_col_async30/2(imag1)
  fir_col_async29/3(real_out2) -> fir_col_async30/3(real2)
  fir_col_async29/4(imag_out2) -> fir_col_async30/4(imag2)
  fir_col_async29/5(real_out3) -> fir_col_async30/5(real3)
  fir_col_async29/6(imag_out3) -> fir_col_async30/6(imag3)
  fir_col_async29/7(real_out4) -> fir_col_async30/7(real4)
  fir_col_async29/8(imag_out4) -> fir_col_async30/8(imag4)
  fir_col_async29/9(real_out5) -> fir_col_async30/9(real5)
  fir_col_async29/10(imag_out5) -> fir_col_async30/10(imag5)
  fir_col_async29/11(real_out6) -> fir_col_async30/11(real6)
  fir_col_async29/12(imag_out6) -> fir_col_async30/12(imag6)
  fir_col_async29/13(real_out7) -> fir_col_async30/13(real7)
  fir_col_async29/14(imag_out7) -> fir_col_async30/14(imag7)
  fir_col_async29/15(real_out8) -> fir_col_async30/15(real8)
  fir_col_async29/16(imag_out8) -> fir_col_async30/16(imag8)
  fir_col_async30/33(real_sum) -> real_sum/31(din30)
  fir_col_async30/34(imag_sum) -> imag_sum/31(din30)
  fir_col_async30/1(real_out1) -> fir_col_async31/1(real1)
  fir_col_async30/2(imag_out1) -> fir_col_async31/2(imag1)
  fir_col_async30/3(real_out2) -> fir_col_async31/3(real2)
  fir_col_async30/4(imag_out2) -> fir_col_async31/4(imag2)
  fir_col_async30/5(real_out3) -> fir_col_async31/5(real3)
  fir_col_async30/6(imag_out3) -> fir_col_async31/6(imag3)
  fir_col_async30/7(real_out4) -> fir_col_async31/7(real4)
  fir_col_async30/8(imag_out4) -> fir_col_async31/8(imag4)
  fir_col_async30/9(real_out5) -> fir_col_async31/9(real5)
  fir_col_async30/10(imag_out5) -> fir_col_async31/10(imag5)
  fir_col_async30/11(real_out6) -> fir_col_async31/11(real6)
  fir_col_async30/12(imag_out6) -> fir_col_async31/12(imag6)
  fir_col_async30/13(real_out7) -> fir_col_async31/13(real7)
  fir_col_async30/14(imag_out7) -> fir_col_async31/14(imag7)
  fir_col_async30/15(real_out8) -> fir_col_async31/15(real8)
  fir_col_async30/16(imag_out8) -> fir_col_async31/16(imag8)
  fir_col_async31/33(real_sum) -> real_sum/32(din31)
  fir_col_async31/34(imag_sum) -> imag_sum/32(din31)
  fir_col_async31/1(real_out1) -> fir_col_async32/1(real1)
  fir_col_async31/2(imag_out1) -> fir_col_async32/2(imag1)
  fir_col_async31/3(real_out2) -> fir_col_async32/3(real2)
  fir_col_async31/4(imag_out2) -> fir_col_async32/4(imag2)
  fir_col_async31/5(real_out3) -> fir_col_async32/5(real3)
  fir_col_async31/6(imag_out3) -> fir_col_async32/6(imag3)
  fir_col_async31/7(real_out4) -> fir_col_async32/7(real4)
  fir_col_async31/8(imag_out4) -> fir_col_async32/8(imag4)
  fir_col_async31/9(real_out5) -> fir_col_async32/9(real5)
  fir_col_async31/10(imag_out5) -> fir_col_async32/10(imag5)
  fir_col_async31/11(real_out6) -> fir_col_async32/11(real6)
  fir_col_async31/12(imag_out6) -> fir_col_async32/12(imag6)
  fir_col_async31/13(real_out7) -> fir_col_async32/13(real7)
  fir_col_async31/14(imag_out7) -> fir_col_async32/14(imag7)
  fir_col_async31/15(real_out8) -> fir_col_async32/15(real8)
  fir_col_async31/16(imag_out8) -> fir_col_async32/16(imag8)
  fir_col_async32/33(real_sum) -> real_sum/33(din32)
  fir_col_async32/34(imag_sum) -> imag_sum/33(din32)
  real_sum/2(dout) -> shift1/1
  imag_sum/2(dout) -> shift2/1
  shift1/1 -> convert1/1
  shift2/1 -> convert2/1
  convert1/1 -> ri_to_c/1
  convert2/1 -> ri_to_c/2
  ri_to_c/1 -> dout/1
  sync_delay/1 -> real_sum/1(sync), imag_sum/1(sync)
  real_sum/1(sync_out) -> sync_out/1
  fir_col_async2/17(real_back_out1) -> fir_col_async1/17(real_back1)
  fir_col_async2/18(imag_back_out1) -> fir_col_async1/18(imag_back1)
  fir_col_async2/19(real_back_out2) -> fir_col_async1/19(real_back2)
  fir_col_async2/20(imag_back_out2) -> fir_col_async1/20(imag_back2)
  fir_col_async2/21(real_back_out3) -> fir_col_async1/21(real_back3)
  fir_col_async2/22(imag_back_out3) -> fir_col_async1/22(imag_back3)
  fir_col_async2/23(real_back_out4) -> fir_col_async1/23(real_back4)
  fir_col_async2/24(imag_back_out4) -> fir_col_async1/24(imag_back4)
  fir_col_async2/25(real_back_out5) -> fir_col_async1/25(real_back5)
  fir_col_async2/26(imag_back_out5) -> fir_col_async1/26(imag_back5)
  fir_col_async2/27(real_back_out6) -> fir_col_async1/27(real_back6)
  fir_col_async2/28(imag_back_out6) -> fir_col_async1/28(imag_back6)
  fir_col_async2/29(real_back_out7) -> fir_col_async1/29(real_back7)
  fir_col_async2/30(imag_back_out7) -> fir_col_async1/30(imag_back7)
  fir_col_async2/31(real_back_out8) -> fir_col_async1/31(real_back8)
  fir_col_async2/32(imag_back_out8) -> fir_col_async1/32(imag_back8)
  fir_col_async3/17(real_back_out1) -> fir_col_async2/17(real_back1)
  fir_col_async3/18(imag_back_out1) -> fir_col_async2/18(imag_back1)
  fir_col_async3/19(real_back_out2) -> fir_col_async2/19(real_back2)
  fir_col_async3/20(imag_back_out2) -> fir_col_async2/20(imag_back2)
  fir_col_async3/21(real_back_out3) -> fir_col_async2/21(real_back3)
  fir_col_async3/22(imag_back_out3) -> fir_col_async2/22(imag_back3)
  fir_col_async3/23(real_back_out4) -> fir_col_async2/23(real_back4)
  fir_col_async3/24(imag_back_out4) -> fir_col_async2/24(imag_back4)
  fir_col_async3/25(real_back_out5) -> fir_col_async2/25(real_back5)
  fir_col_async3/26(imag_back_out5) -> fir_col_async2/26(imag_back5)
  fir_col_async3/27(real_back_out6) -> fir_col_async2/27(real_back6)
  fir_col_async3/28(imag_back_out6) -> fir_col_async2/28(imag_back6)
  fir_col_async3/29(real_back_out7) -> fir_col_async2/29(real_back7)
  fir_col_async3/30(imag_back_out7) -> fir_col_async2/30(imag_back7)
  fir_col_async3/31(real_back_out8) -> fir_col_async2/31(real_back8)
  fir_col_async3/32(imag_back_out8) -> fir_col_async2/32(imag_back8)
  fir_col_async4/17(real_back_out1) -> fir_col_async3/17(real_back1)
  fir_col_async4/18(imag_back_out1) -> fir_col_async3/18(imag_back1)
  fir_col_async4/19(real_back_out2) -> fir_col_async3/19(real_back2)
  fir_col_async4/20(imag_back_out2) -> fir_col_async3/20(imag_back2)
  fir_col_async4/21(real_back_out3) -> fir_col_async3/21(real_back3)
  fir_col_async4/22(imag_back_out3) -> fir_col_async3/22(imag_back3)
  fir_col_async4/23(real_back_out4) -> fir_col_async3/23(real_back4)
  fir_col_async4/24(imag_back_out4) -> fir_col_async3/24(imag_back4)
  fir_col_async4/25(real_back_out5) -> fir_col_async3/25(real_back5)
  fir_col_async4/26(imag_back_out5) -> fir_col_async3/26(imag_back5)
  fir_col_async4/27(real_back_out6) -> fir_col_async3/27(real_back6)
  fir_col_async4/28(imag_back_out6) -> fir_col_async3/28(imag_back6)
  fir_col_async4/29(real_back_out7) -> fir_col_async3/29(real_back7)
  fir_col_async4/30(imag_back_out7) -> fir_col_async3/30(imag_back7)
  fir_col_async4/31(real_back_out8) -> fir_col_async3/31(real_back8)
  fir_col_async4/32(imag_back_out8) -> fir_col_async3/32(imag_back8)
  fir_col_async5/17(real_back_out1) -> fir_col_async4/17(real_back1)
  fir_col_async5/18(imag_back_out1) -> fir_col_async4/18(imag_back1)
  fir_col_async5/19(real_back_out2) -> fir_col_async4/19(real_back2)
  fir_col_async5/20(imag_back_out2) -> fir_col_async4/20(imag_back2)
  fir_col_async5/21(real_back_out3) -> fir_col_async4/21(real_back3)
  fir_col_async5/22(imag_back_out3) -> fir_col_async4/22(imag_back3)
  fir_col_async5/23(real_back_out4) -> fir_col_async4/23(real_back4)
  fir_col_async5/24(imag_back_out4) -> fir_col_async4/24(imag_back4)
  fir_col_async5/25(real_back_out5) -> fir_col_async4/25(real_back5)
  fir_col_async5/26(imag_back_out5) -> fir_col_async4/26(imag_back5)
  fir_col_async5/27(real_back_out6) -> fir_col_async4/27(real_back6)
  fir_col_async5/28(imag_back_out6) -> fir_col_async4/28(imag_back6)
  fir_col_async5/29(real_back_out7) -> fir_col_async4/29(real_back7)
  fir_col_async5/30(imag_back_out7) -> fir_col_async4/30(imag_back7)
  fir_col_async5/31(real_back_out8) -> fir_col_async4/31(real_back8)
  fir_col_async5/32(imag_back_out8) -> fir_col_async4/32(imag_back8)
  fir_col_async6/17(real_back_out1) -> fir_col_async5/17(real_back1)
  fir_col_async6/18(imag_back_out1) -> fir_col_async5/18(imag_back1)
  fir_col_async6/19(real_back_out2) -> fir_col_async5/19(real_back2)
  fir_col_async6/20(imag_back_out2) -> fir_col_async5/20(imag_back2)
  fir_col_async6/21(real_back_out3) -> fir_col_async5/21(real_back3)
  fir_col_async6/22(imag_back_out3) -> fir_col_async5/22(imag_back3)
  fir_col_async6/23(real_back_out4) -> fir_col_async5/23(real_back4)
  fir_col_async6/24(imag_back_out4) -> fir_col_async5/24(imag_back4)
  fir_col_async6/25(real_back_out5) -> fir_col_async5/25(real_back5)
  fir_col_async6/26(imag_back_out5) -> fir_col_async5/26(imag_back5)
  fir_col_async6/27(real_back_out6) -> fir_col_async5/27(real_back6)
  fir_col_async6/28(imag_back_out6) -> fir_col_async5/28(imag_back6)
  fir_col_async6/29(real_back_out7) -> fir_col_async5/29(real_back7)
  fir_col_async6/30(imag_back_out7) -> fir_col_async5/30(imag_back7)
  fir_col_async6/31(real_back_out8) -> fir_col_async5/31(real_back8)
  fir_col_async6/32(imag_back_out8) -> fir_col_async5/32(imag_back8)
  fir_col_async7/17(real_back_out1) -> fir_col_async6/17(real_back1)
  fir_col_async7/18(imag_back_out1) -> fir_col_async6/18(imag_back1)
  fir_col_async7/19(real_back_out2) -> fir_col_async6/19(real_back2)
  fir_col_async7/20(imag_back_out2) -> fir_col_async6/20(imag_back2)
  fir_col_async7/21(real_back_out3) -> fir_col_async6/21(real_back3)
  fir_col_async7/22(imag_back_out3) -> fir_col_async6/22(imag_back3)
  fir_col_async7/23(real_back_out4) -> fir_col_async6/23(real_back4)
  fir_col_async7/24(imag_back_out4) -> fir_col_async6/24(imag_back4)
  fir_col_async7/25(real_back_out5) -> fir_col_async6/25(real_back5)
  fir_col_async7/26(imag_back_out5) -> fir_col_async6/26(imag_back5)
  fir_col_async7/27(real_back_out6) -> fir_col_async6/27(real_back6)
  fir_col_async7/28(imag_back_out6) -> fir_col_async6/28(imag_back6)
  fir_col_async7/29(real_back_out7) -> fir_col_async6/29(real_back7)
  fir_col_async7/30(imag_back_out7) -> fir_col_async6/30(imag_back7)
  fir_col_async7/31(real_back_out8) -> fir_col_async6/31(real_back8)
  fir_col_async7/32(imag_back_out8) -> fir_col_async6/32(imag_back8)
  fir_col_async8/17(real_back_out1) -> fir_col_async7/17(real_back1)
  fir_col_async8/18(imag_back_out1) -> fir_col_async7/18(imag_back1)
  fir_col_async8/19(real_back_out2) -> fir_col_async7/19(real_back2)
  fir_col_async8/20(imag_back_out2) -> fir_col_async7/20(imag_back2)
  fir_col_async8/21(real_back_out3) -> fir_col_async7/21(real_back3)
  fir_col_async8/22(imag_back_out3) -> fir_col_async7/22(imag_back3)
  fir_col_async8/23(real_back_out4) -> fir_col_async7/23(real_back4)
  fir_col_async8/24(imag_back_out4) -> fir_col_async7/24(imag_back4)
  fir_col_async8/25(real_back_out5) -> fir_col_async7/25(real_back5)
  fir_col_async8/26(imag_back_out5) -> fir_col_async7/26(imag_back5)
  fir_col_async8/27(real_back_out6) -> fir_col_async7/27(real_back6)
  fir_col_async8/28(imag_back_out6) -> fir_col_async7/28(imag_back6)
  fir_col_async8/29(real_back_out7) -> fir_col_async7/29(real_back7)
  fir_col_async8/30(imag_back_out7) -> fir_col_async7/30(imag_back7)
  fir_col_async8/31(real_back_out8) -> fir_col_async7/31(real_back8)
  fir_col_async8/32(imag_back_out8) -> fir_col_async7/32(imag_back8)
  fir_col_async9/17(real_back_out1) -> fir_col_async8/17(real_back1)
  fir_col_async9/18(imag_back_out1) -> fir_col_async8/18(imag_back1)
  fir_col_async9/19(real_back_out2) -> fir_col_async8/19(real_back2)
  fir_col_async9/20(imag_back_out2) -> fir_col_async8/20(imag_back2)
  fir_col_async9/21(real_back_out3) -> fir_col_async8/21(real_back3)
  fir_col_async9/22(imag_back_out3) -> fir_col_async8/22(imag_back3)
  fir_col_async9/23(real_back_out4) -> fir_col_async8/23(real_back4)
  fir_col_async9/24(imag_back_out4) -> fir_col_async8/24(imag_back4)
  fir_col_async9/25(real_back_out5) -> fir_col_async8/25(real_back5)
  fir_col_async9/26(imag_back_out5) -> fir_col_async8/26(imag_back5)
  fir_col_async9/27(real_back_out6) -> fir_col_async8/27(real_back6)
  fir_col_async9/28(imag_back_out6) -> fir_col_async8/28(imag_back6)
  fir_col_async9/29(real_back_out7) -> fir_col_async8/29(real_back7)
  fir_col_async9/30(imag_back_out7) -> fir_col_async8/30(imag_back7)
  fir_col_async9/31(real_back_out8) -> fir_col_async8/31(real_back8)
  fir_col_async9/32(imag_back_out8) -> fir_col_async8/32(imag_back8)
  fir_col_async10/17(real_back_out1) -> fir_col_async9/17(real_back1)
  fir_col_async10/18(imag_back_out1) -> fir_col_async9/18(imag_back1)
  fir_col_async10/19(real_back_out2) -> fir_col_async9/19(real_back2)
  fir_col_async10/20(imag_back_out2) -> fir_col_async9/20(imag_back2)
  fir_col_async10/21(real_back_out3) -> fir_col_async9/21(real_back3)
  fir_col_async10/22(imag_back_out3) -> fir_col_async9/22(imag_back3)
  fir_col_async10/23(real_back_out4) -> fir_col_async9/23(real_back4)
  fir_col_async10/24(imag_back_out4) -> fir_col_async9/24(imag_back4)
  fir_col_async10/25(real_back_out5) -> fir_col_async9/25(real_back5)
  fir_col_async10/26(imag_back_out5) -> fir_col_async9/26(imag_back5)
  fir_col_async10/27(real_back_out6) -> fir_col_async9/27(real_back6)
  fir_col_async10/28(imag_back_out6) -> fir_col_async9/28(imag_back6)
  fir_col_async10/29(real_back_out7) -> fir_col_async9/29(real_back7)
  fir_col_async10/30(imag_back_out7) -> fir_col_async9/30(imag_back7)
  fir_col_async10/31(real_back_out8) -> fir_col_async9/31(real_back8)
  fir_col_async10/32(imag_back_out8) -> fir_col_async9/32(imag_back8)
  fir_col_async11/17(real_back_out1) -> fir_col_async10/17(real_back1)
  fir_col_async11/18(imag_back_out1) -> fir_col_async10/18(imag_back1)
  fir_col_async11/19(real_back_out2) -> fir_col_async10/19(real_back2)
  fir_col_async11/20(imag_back_out2) -> fir_col_async10/20(imag_back2)
  fir_col_async11/21(real_back_out3) -> fir_col_async10/21(real_back3)
  fir_col_async11/22(imag_back_out3) -> fir_col_async10/22(imag_back3)
  fir_col_async11/23(real_back_out4) -> fir_col_async10/23(real_back4)
  fir_col_async11/24(imag_back_out4) -> fir_col_async10/24(imag_back4)
  fir_col_async11/25(real_back_out5) -> fir_col_async10/25(real_back5)
  fir_col_async11/26(imag_back_out5) -> fir_col_async10/26(imag_back5)
  fir_col_async11/27(real_back_out6) -> fir_col_async10/27(real_back6)
  fir_col_async11/28(imag_back_out6) -> fir_col_async10/28(imag_back6)
  fir_col_async11/29(real_back_out7) -> fir_col_async10/29(real_back7)
  fir_col_async11/30(imag_back_out7) -> fir_col_async10/30(imag_back7)
  fir_col_async11/31(real_back_out8) -> fir_col_async10/31(real_back8)
  fir_col_async11/32(imag_back_out8) -> fir_col_async10/32(imag_back8)
  fir_col_async12/17(real_back_out1) -> fir_col_async11/17(real_back1)
  fir_col_async12/18(imag_back_out1) -> fir_col_async11/18(imag_back1)
  fir_col_async12/19(real_back_out2) -> fir_col_async11/19(real_back2)
  fir_col_async12/20(imag_back_out2) -> fir_col_async11/20(imag_back2)
  fir_col_async12/21(real_back_out3) -> fir_col_async11/21(real_back3)
  fir_col_async12/22(imag_back_out3) -> fir_col_async11/22(imag_back3)
  fir_col_async12/23(real_back_out4) -> fir_col_async11/23(real_back4)
  fir_col_async12/24(imag_back_out4) -> fir_col_async11/24(imag_back4)
  fir_col_async12/25(real_back_out5) -> fir_col_async11/25(real_back5)
  fir_col_async12/26(imag_back_out5) -> fir_col_async11/26(imag_back5)
  fir_col_async12/27(real_back_out6) -> fir_col_async11/27(real_back6)
  fir_col_async12/28(imag_back_out6) -> fir_col_async11/28(imag_back6)
  fir_col_async12/29(real_back_out7) -> fir_col_async11/29(real_back7)
  fir_col_async12/30(imag_back_out7) -> fir_col_async11/30(imag_back7)
  fir_col_async12/31(real_back_out8) -> fir_col_async11/31(real_back8)
  fir_col_async12/32(imag_back_out8) -> fir_col_async11/32(imag_back8)
  fir_col_async13/17(real_back_out1) -> fir_col_async12/17(real_back1)
  fir_col_async13/18(imag_back_out1) -> fir_col_async12/18(imag_back1)
  fir_col_async13/19(real_back_out2) -> fir_col_async12/19(real_back2)
  fir_col_async13/20(imag_back_out2) -> fir_col_async12/20(imag_back2)
  fir_col_async13/21(real_back_out3) -> fir_col_async12/21(real_back3)
  fir_col_async13/22(imag_back_out3) -> fir_col_async12/22(imag_back3)
  fir_col_async13/23(real_back_out4) -> fir_col_async12/23(real_back4)
  fir_col_async13/24(imag_back_out4) -> fir_col_async12/24(imag_back4)
  fir_col_async13/25(real_back_out5) -> fir_col_async12/25(real_back5)
  fir_col_async13/26(imag_back_out5) -> fir_col_async12/26(imag_back5)
  fir_col_async13/27(real_back_out6) -> fir_col_async12/27(real_back6)
  fir_col_async13/28(imag_back_out6) -> fir_col_async12/28(imag_back6)
  fir_col_async13/29(real_back_out7) -> fir_col_async12/29(real_back7)
  fir_col_async13/30(imag_back_out7) -> fir_col_async12/30(imag_back7)
  fir_col_async13/31(real_back_out8) -> fir_col_async12/31(real_back8)
  fir_col_async13/32(imag_back_out8) -> fir_col_async12/32(imag_back8)
  fir_col_async14/17(real_back_out1) -> fir_col_async13/17(real_back1)
  fir_col_async14/18(imag_back_out1) -> fir_col_async13/18(imag_back1)
  fir_col_async14/19(real_back_out2) -> fir_col_async13/19(real_back2)
  fir_col_async14/20(imag_back_out2) -> fir_col_async13/20(imag_back2)
  fir_col_async14/21(real_back_out3) -> fir_col_async13/21(real_back3)
  fir_col_async14/22(imag_back_out3) -> fir_col_async13/22(imag_back3)
  fir_col_async14/23(real_back_out4) -> fir_col_async13/23(real_back4)
  fir_col_async14/24(imag_back_out4) -> fir_col_async13/24(imag_back4)
  fir_col_async14/25(real_back_out5) -> fir_col_async13/25(real_back5)
  fir_col_async14/26(imag_back_out5) -> fir_col_async13/26(imag_back5)
  fir_col_async14/27(real_back_out6) -> fir_col_async13/27(real_back6)
  fir_col_async14/28(imag_back_out6) -> fir_col_async13/28(imag_back6)
  fir_col_async14/29(real_back_out7) -> fir_col_async13/29(real_back7)
  fir_col_async14/30(imag_back_out7) -> fir_col_async13/30(imag_back7)
  fir_col_async14/31(real_back_out8) -> fir_col_async13/31(real_back8)
  fir_col_async14/32(imag_back_out8) -> fir_col_async13/32(imag_back8)
  fir_col_async15/17(real_back_out1) -> fir_col_async14/17(real_back1)
  fir_col_async15/18(imag_back_out1) -> fir_col_async14/18(imag_back1)
  fir_col_async15/19(real_back_out2) -> fir_col_async14/19(real_back2)
  fir_col_async15/20(imag_back_out2) -> fir_col_async14/20(imag_back2)
  fir_col_async15/21(real_back_out3) -> fir_col_async14/21(real_back3)
  fir_col_async15/22(imag_back_out3) -> fir_col_async14/22(imag_back3)
  fir_col_async15/23(real_back_out4) -> fir_col_async14/23(real_back4)
  fir_col_async15/24(imag_back_out4) -> fir_col_async14/24(imag_back4)
  fir_col_async15/25(real_back_out5) -> fir_col_async14/25(real_back5)
  fir_col_async15/26(imag_back_out5) -> fir_col_async14/26(imag_back5)
  fir_col_async15/27(real_back_out6) -> fir_col_async14/27(real_back6)
  fir_col_async15/28(imag_back_out6) -> fir_col_async14/28(imag_back6)
  fir_col_async15/29(real_back_out7) -> fir_col_async14/29(real_back7)
  fir_col_async15/30(imag_back_out7) -> fir_col_async14/30(imag_back7)
  fir_col_async15/31(real_back_out8) -> fir_col_async14/31(real_back8)
  fir_col_async15/32(imag_back_out8) -> fir_col_async14/32(imag_back8)
  fir_col_async16/17(real_back_out1) -> fir_col_async15/17(real_back1)
  fir_col_async16/18(imag_back_out1) -> fir_col_async15/18(imag_back1)
  fir_col_async16/19(real_back_out2) -> fir_col_async15/19(real_back2)
  fir_col_async16/20(imag_back_out2) -> fir_col_async15/20(imag_back2)
  fir_col_async16/21(real_back_out3) -> fir_col_async15/21(real_back3)
  fir_col_async16/22(imag_back_out3) -> fir_col_async15/22(imag_back3)
  fir_col_async16/23(real_back_out4) -> fir_col_async15/23(real_back4)
  fir_col_async16/24(imag_back_out4) -> fir_col_async15/24(imag_back4)
  fir_col_async16/25(real_back_out5) -> fir_col_async15/25(real_back5)
  fir_col_async16/26(imag_back_out5) -> fir_col_async15/26(imag_back5)
  fir_col_async16/27(real_back_out6) -> fir_col_async15/27(real_back6)
  fir_col_async16/28(imag_back_out6) -> fir_col_async15/28(imag_back6)
  fir_col_async16/29(real_back_out7) -> fir_col_async15/29(real_back7)
  fir_col_async16/30(imag_back_out7) -> fir_col_async15/30(imag_back7)
  fir_col_async16/31(real_back_out8) -> fir_col_async15/31(real_back8)
  fir_col_async16/32(imag_back_out8) -> fir_col_async15/32(imag_back8)
  fir_col_async17/17(real_back_out1) -> fir_col_async16/17(real_back1)
  fir_col_async17/18(imag_back_out1) -> fir_col_async16/18(imag_back1)
  fir_col_async17/19(real_back_out2) -> fir_col_async16/19(real_back2)
  fir_col_async17/20(imag_back_out2) -> fir_col_async16/20(imag_back2)
  fir_col_async17/21(real_back_out3) -> fir_col_async16/21(real_back3)
  fir_col_async17/22(imag_back_out3) -> fir_col_async16/22(imag_back3)
  fir_col_async17/23(real_back_out4) -> fir_col_async16/23(real_back4)
  fir_col_async17/24(imag_back_out4) -> fir_col_async16/24(imag_back4)
  fir_col_async17/25(real_back_out5) -> fir_col_async16/25(real_back5)
  fir_col_async17/26(imag_back_out5) -> fir_col_async16/26(imag_back5)
  fir_col_async17/27(real_back_out6) -> fir_col_async16/27(real_back6)
  fir_col_async17/28(imag_back_out6) -> fir_col_async16/28(imag_back6)
  fir_col_async17/29(real_back_out7) -> fir_col_async16/29(real_back7)
  fir_col_async17/30(imag_back_out7) -> fir_col_async16/30(imag_back7)
  fir_col_async17/31(real_back_out8) -> fir_col_async16/31(real_back8)
  fir_col_async17/32(imag_back_out8) -> fir_col_async16/32(imag_back8)
  fir_col_async18/17(real_back_out1) -> fir_col_async17/17(real_back1)
  fir_col_async18/18(imag_back_out1) -> fir_col_async17/18(imag_back1)
  fir_col_async18/19(real_back_out2) -> fir_col_async17/19(real_back2)
  fir_col_async18/20(imag_back_out2) -> fir_col_async17/20(imag_back2)
  fir_col_async18/21(real_back_out3) -> fir_col_async17/21(real_back3)
  fir_col_async18/22(imag_back_out3) -> fir_col_async17/22(imag_back3)
  fir_col_async18/23(real_back_out4) -> fir_col_async17/23(real_back4)
  fir_col_async18/24(imag_back_out4) -> fir_col_async17/24(imag_back4)
  fir_col_async18/25(real_back_out5) -> fir_col_async17/25(real_back5)
  fir_col_async18/26(imag_back_out5) -> fir_col_async17/26(imag_back5)
  fir_col_async18/27(real_back_out6) -> fir_col_async17/27(real_back6)
  fir_col_async18/28(imag_back_out6) -> fir_col_async17/28(imag_back6)
  fir_col_async18/29(real_back_out7) -> fir_col_async17/29(real_back7)
  fir_col_async18/30(imag_back_out7) -> fir_col_async17/30(imag_back7)
  fir_col_async18/31(real_back_out8) -> fir_col_async17/31(real_back8)
  fir_col_async18/32(imag_back_out8) -> fir_col_async17/32(imag_back8)
  fir_col_async19/17(real_back_out1) -> fir_col_async18/17(real_back1)
  fir_col_async19/18(imag_back_out1) -> fir_col_async18/18(imag_back1)
  fir_col_async19/19(real_back_out2) -> fir_col_async18/19(real_back2)
  fir_col_async19/20(imag_back_out2) -> fir_col_async18/20(imag_back2)
  fir_col_async19/21(real_back_out3) -> fir_col_async18/21(real_back3)
  fir_col_async19/22(imag_back_out3) -> fir_col_async18/22(imag_back3)
  fir_col_async19/23(real_back_out4) -> fir_col_async18/23(real_back4)
  fir_col_async19/24(imag_back_out4) -> fir_col_async18/24(imag_back4)
  fir_col_async19/25(real_back_out5) -> fir_col_async18/25(real_back5)
  fir_col_async19/26(imag_back_out5) -> fir_col_async18/26(imag_back5)
  fir_col_async19/27(real_back_out6) -> fir_col_async18/27(real_back6)
  fir_col_async19/28(imag_back_out6) -> fir_col_async18/28(imag_back6)
  fir_col_async19/29(real_back_out7) -> fir_col_async18/29(real_back7)
  fir_col_async19/30(imag_back_out7) -> fir_col_async18/30(imag_back7)
  fir_col_async19/31(real_back_out8) -> fir_col_async18/31(real_back8)
  fir_col_async19/32(imag_back_out8) -> fir_col_async18/32(imag_back8)
  fir_col_async20/17(real_back_out1) -> fir_col_async19/17(real_back1)
  fir_col_async20/18(imag_back_out1) -> fir_col_async19/18(imag_back1)
  fir_col_async20/19(real_back_out2) -> fir_col_async19/19(real_back2)
  fir_col_async20/20(imag_back_out2) -> fir_col_async19/20(imag_back2)
  fir_col_async20/21(real_back_out3) -> fir_col_async19/21(real_back3)
  fir_col_async20/22(imag_back_out3) -> fir_col_async19/22(imag_back3)
  fir_col_async20/23(real_back_out4) -> fir_col_async19/23(real_back4)
  fir_col_async20/24(imag_back_out4) -> fir_col_async19/24(imag_back4)
  fir_col_async20/25(real_back_out5) -> fir_col_async19/25(real_back5)
  fir_col_async20/26(imag_back_out5) -> fir_col_async19/26(imag_back5)
  fir_col_async20/27(real_back_out6) -> fir_col_async19/27(real_back6)
  fir_col_async20/28(imag_back_out6) -> fir_col_async19/28(imag_back6)
  fir_col_async20/29(real_back_out7) -> fir_col_async19/29(real_back7)
  fir_col_async20/30(imag_back_out7) -> fir_col_async19/30(imag_back7)
  fir_col_async20/31(real_back_out8) -> fir_col_async19/31(real_back8)
  fir_col_async20/32(imag_back_out8) -> fir_col_async19/32(imag_back8)
  fir_col_async21/17(real_back_out1) -> fir_col_async20/17(real_back1)
  fir_col_async21/18(imag_back_out1) -> fir_col_async20/18(imag_back1)
  fir_col_async21/19(real_back_out2) -> fir_col_async20/19(real_back2)
  fir_col_async21/20(imag_back_out2) -> fir_col_async20/20(imag_back2)
  fir_col_async21/21(real_back_out3) -> fir_col_async20/21(real_back3)
  fir_col_async21/22(imag_back_out3) -> fir_col_async20/22(imag_back3)
  fir_col_async21/23(real_back_out4) -> fir_col_async20/23(real_back4)
  fir_col_async21/24(imag_back_out4) -> fir_col_async20/24(imag_back4)
  fir_col_async21/25(real_back_out5) -> fir_col_async20/25(real_back5)
  fir_col_async21/26(imag_back_out5) -> fir_col_async20/26(imag_back5)
  fir_col_async21/27(real_back_out6) -> fir_col_async20/27(real_back6)
  fir_col_async21/28(imag_back_out6) -> fir_col_async20/28(imag_back6)
  fir_col_async21/29(real_back_out7) -> fir_col_async20/29(real_back7)
  fir_col_async21/30(imag_back_out7) -> fir_col_async20/30(imag_back7)
  fir_col_async21/31(real_back_out8) -> fir_col_async20/31(real_back8)
  fir_col_async21/32(imag_back_out8) -> fir_col_async20/32(imag_back8)
  fir_col_async22/17(real_back_out1) -> fir_col_async21/17(real_back1)
  fir_col_async22/18(imag_back_out1) -> fir_col_async21/18(imag_back1)
  fir_col_async22/19(real_back_out2) -> fir_col_async21/19(real_back2)
  fir_col_async22/20(imag_back_out2) -> fir_col_async21/20(imag_back2)
  fir_col_async22/21(real_back_out3) -> fir_col_async21/21(real_back3)
  fir_col_async22/22(imag_back_out3) -> fir_col_async21/22(imag_back3)
  fir_col_async22/23(real_back_out4) -> fir_col_async21/23(real_back4)
  fir_col_async22/24(imag_back_out4) -> fir_col_async21/24(imag_back4)
  fir_col_async22/25(real_back_out5) -> fir_col_async21/25(real_back5)
  fir_col_async22/26(imag_back_out5) -> fir_col_async21/26(imag_back5)
  fir_col_async22/27(real_back_out6) -> fir_col_async21/27(real_back6)
  fir_col_async22/28(imag_back_out6) -> fir_col_async21/28(imag_back6)
  fir_col_async22/29(real_back_out7) -> fir_col_async21/29(real_back7)
  fir_col_async22/30(imag_back_out7) -> fir_col_async21/30(imag_back7)
  fir_col_async22/31(real_back_out8) -> fir_col_async21/31(real_back8)
  fir_col_async22/32(imag_back_out8) -> fir_col_async21/32(imag_back8)
  fir_col_async23/17(real_back_out1) -> fir_col_async22/17(real_back1)
  fir_col_async23/18(imag_back_out1) -> fir_col_async22/18(imag_back1)
  fir_col_async23/19(real_back_out2) -> fir_col_async22/19(real_back2)
  fir_col_async23/20(imag_back_out2) -> fir_col_async22/20(imag_back2)
  fir_col_async23/21(real_back_out3) -> fir_col_async22/21(real_back3)
  fir_col_async23/22(imag_back_out3) -> fir_col_async22/22(imag_back3)
  fir_col_async23/23(real_back_out4) -> fir_col_async22/23(real_back4)
  fir_col_async23/24(imag_back_out4) -> fir_col_async22/24(imag_back4)
  fir_col_async23/25(real_back_out5) -> fir_col_async22/25(real_back5)
  fir_col_async23/26(imag_back_out5) -> fir_col_async22/26(imag_back5)
  fir_col_async23/27(real_back_out6) -> fir_col_async22/27(real_back6)
  fir_col_async23/28(imag_back_out6) -> fir_col_async22/28(imag_back6)
  fir_col_async23/29(real_back_out7) -> fir_col_async22/29(real_back7)
  fir_col_async23/30(imag_back_out7) -> fir_col_async22/30(imag_back7)
  fir_col_async23/31(real_back_out8) -> fir_col_async22/31(real_back8)
  fir_col_async23/32(imag_back_out8) -> fir_col_async22/32(imag_back8)
  fir_col_async24/17(real_back_out1) -> fir_col_async23/17(real_back1)
  fir_col_async24/18(imag_back_out1) -> fir_col_async23/18(imag_back1)
  fir_col_async24/19(real_back_out2) -> fir_col_async23/19(real_back2)
  fir_col_async24/20(imag_back_out2) -> fir_col_async23/20(imag_back2)
  fir_col_async24/21(real_back_out3) -> fir_col_async23/21(real_back3)
  fir_col_async24/22(imag_back_out3) -> fir_col_async23/22(imag_back3)
  fir_col_async24/23(real_back_out4) -> fir_col_async23/23(real_back4)
  fir_col_async24/24(imag_back_out4) -> fir_col_async23/24(imag_back4)
  fir_col_async24/25(real_back_out5) -> fir_col_async23/25(real_back5)
  fir_col_async24/26(imag_back_out5) -> fir_col_async23/26(imag_back5)
  fir_col_async24/27(real_back_out6) -> fir_col_async23/27(real_back6)
  fir_col_async24/28(imag_back_out6) -> fir_col_async23/28(imag_back6)
  fir_col_async24/29(real_back_out7) -> fir_col_async23/29(real_back7)
  fir_col_async24/30(imag_back_out7) -> fir_col_async23/30(imag_back7)
  fir_col_async24/31(real_back_out8) -> fir_col_async23/31(real_back8)
  fir_col_async24/32(imag_back_out8) -> fir_col_async23/32(imag_back8)
  fir_col_async25/17(real_back_out1) -> fir_col_async24/17(real_back1)
  fir_col_async25/18(imag_back_out1) -> fir_col_async24/18(imag_back1)
  fir_col_async25/19(real_back_out2) -> fir_col_async24/19(real_back2)
  fir_col_async25/20(imag_back_out2) -> fir_col_async24/20(imag_back2)
  fir_col_async25/21(real_back_out3) -> fir_col_async24/21(real_back3)
  fir_col_async25/22(imag_back_out3) -> fir_col_async24/22(imag_back3)
  fir_col_async25/23(real_back_out4) -> fir_col_async24/23(real_back4)
  fir_col_async25/24(imag_back_out4) -> fir_col_async24/24(imag_back4)
  fir_col_async25/25(real_back_out5) -> fir_col_async24/25(real_back5)
  fir_col_async25/26(imag_back_out5) -> fir_col_async24/26(imag_back5)
  fir_col_async25/27(real_back_out6) -> fir_col_async24/27(real_back6)
  fir_col_async25/28(imag_back_out6) -> fir_col_async24/28(imag_back6)
  fir_col_async25/29(real_back_out7) -> fir_col_async24/29(real_back7)
  fir_col_async25/30(imag_back_out7) -> fir_col_async24/30(imag_back7)
  fir_col_async25/31(real_back_out8) -> fir_col_async24/31(real_back8)
  fir_col_async25/32(imag_back_out8) -> fir_col_async24/32(imag_back8)
  fir_col_async26/17(real_back_out1) -> fir_col_async25/17(real_back1)
  fir_col_async26/18(imag_back_out1) -> fir_col_async25/18(imag_back1)
  fir_col_async26/19(real_back_out2) -> fir_col_async25/19(real_back2)
  fir_col_async26/20(imag_back_out2) -> fir_col_async25/20(imag_back2)
  fir_col_async26/21(real_back_out3) -> fir_col_async25/21(real_back3)
  fir_col_async26/22(imag_back_out3) -> fir_col_async25/22(imag_back3)
  fir_col_async26/23(real_back_out4) -> fir_col_async25/23(real_back4)
  fir_col_async26/24(imag_back_out4) -> fir_col_async25/24(imag_back4)
  fir_col_async26/25(real_back_out5) -> fir_col_async25/25(real_back5)
  fir_col_async26/26(imag_back_out5) -> fir_col_async25/26(imag_back5)
  fir_col_async26/27(real_back_out6) -> fir_col_async25/27(real_back6)
  fir_col_async26/28(imag_back_out6) -> fir_col_async25/28(imag_back6)
  fir_col_async26/29(real_back_out7) -> fir_col_async25/29(real_back7)
  fir_col_async26/30(imag_back_out7) -> fir_col_async25/30(imag_back7)
  fir_col_async26/31(real_back_out8) -> fir_col_async25/31(real_back8)
  fir_col_async26/32(imag_back_out8) -> fir_col_async25/32(imag_back8)
  fir_col_async27/17(real_back_out1) -> fir_col_async26/17(real_back1)
  fir_col_async27/18(imag_back_out1) -> fir_col_async26/18(imag_back1)
  fir_col_async27/19(real_back_out2) -> fir_col_async26/19(real_back2)
  fir_col_async27/20(imag_back_out2) -> fir_col_async26/20(imag_back2)
  fir_col_async27/21(real_back_out3) -> fir_col_async26/21(real_back3)
  fir_col_async27/22(imag_back_out3) -> fir_col_async26/22(imag_back3)
  fir_col_async27/23(real_back_out4) -> fir_col_async26/23(real_back4)
  fir_col_async27/24(imag_back_out4) -> fir_col_async26/24(imag_back4)
  fir_col_async27/25(real_back_out5) -> fir_col_async26/25(real_back5)
  fir_col_async27/26(imag_back_out5) -> fir_col_async26/26(imag_back5)
  fir_col_async27/27(real_back_out6) -> fir_col_async26/27(real_back6)
  fir_col_async27/28(imag_back_out6) -> fir_col_async26/28(imag_back6)
  fir_col_async27/29(real_back_out7) -> fir_col_async26/29(real_back7)
  fir_col_async27/30(imag_back_out7) -> fir_col_async26/30(imag_back7)
  fir_col_async27/31(real_back_out8) -> fir_col_async26/31(real_back8)
  fir_col_async27/32(imag_back_out8) -> fir_col_async26/32(imag_back8)
  fir_col_async28/17(real_back_out1) -> fir_col_async27/17(real_back1)
  fir_col_async28/18(imag_back_out1) -> fir_col_async27/18(imag_back1)
  fir_col_async28/19(real_back_out2) -> fir_col_async27/19(real_back2)
  fir_col_async28/20(imag_back_out2) -> fir_col_async27/20(imag_back2)
  fir_col_async28/21(real_back_out3) -> fir_col_async27/21(real_back3)
  fir_col_async28/22(imag_back_out3) -> fir_col_async27/22(imag_back3)
  fir_col_async28/23(real_back_out4) -> fir_col_async27/23(real_back4)
  fir_col_async28/24(imag_back_out4) -> fir_col_async27/24(imag_back4)
  fir_col_async28/25(real_back_out5) -> fir_col_async27/25(real_back5)
  fir_col_async28/26(imag_back_out5) -> fir_col_async27/26(imag_back5)
  fir_col_async28/27(real_back_out6) -> fir_col_async27/27(real_back6)
  fir_col_async28/28(imag_back_out6) -> fir_col_async27/28(imag_back6)
  fir_col_async28/29(real_back_out7) -> fir_col_async27/29(real_back7)
  fir_col_async28/30(imag_back_out7) -> fir_col_async27/30(imag_back7)
  fir_col_async28/31(real_back_out8) -> fir_col_async27/31(real_back8)
  fir_col_async28/32(imag_back_out8) -> fir_col_async27/32(imag_back8)
  fir_col_async29/17(real_back_out1) -> fir_col_async28/17(real_back1)
  fir_col_async29/18(imag_back_out1) -> fir_col_async28/18(imag_back1)
  fir_col_async29/19(real_back_out2) -> fir_col_async28/19(real_back2)
  fir_col_async29/20(imag_back_out2) -> fir_col_async28/20(imag_back2)
  fir_col_async29/21(real_back_out3) -> fir_col_async28/21(real_back3)
  fir_col_async29/22(imag_back_out3) -> fir_col_async28/22(imag_back3)
  fir_col_async29/23(real_back_out4) -> fir_col_async28/23(real_back4)
  fir_col_async29/24(imag_back_out4) -> fir_col_async28/24(imag_back4)
  fir_col_async29/25(real_back_out5) -> fir_col_async28/25(real_back5)
  fir_col_async29/26(imag_back_out5) -> fir_col_async28/26(imag_back5)
  fir_col_async29/27(real_back_out6) -> fir_col_async28/27(real_back6)
  fir_col_async29/28(imag_back_out6) -> fir_col_async28/28(imag_back6)
  fir_col_async29/29(real_back_out7) -> fir_col_async28/29(real_back7)
  fir_col_async29/30(imag_back_out7) -> fir_col_async28/30(imag_back7)
  fir_col_async29/31(real_back_out8) -> fir_col_async28/31(real_back8)
  fir_col_async29/32(imag_back_out8) -> fir_col_async28/32(imag_back8)
  fir_col_async30/17(real_back_out1) -> fir_col_async29/17(real_back1)
  fir_col_async30/18(imag_back_out1) -> fir_col_async29/18(imag_back1)
  fir_col_async30/19(real_back_out2) -> fir_col_async29/19(real_back2)
  fir_col_async30/20(imag_back_out2) -> fir_col_async29/20(imag_back2)
  fir_col_async30/21(real_back_out3) -> fir_col_async29/21(real_back3)
  fir_col_async30/22(imag_back_out3) -> fir_col_async29/22(imag_back3)
  fir_col_async30/23(real_back_out4) -> fir_col_async29/23(real_back4)
  fir_col_async30/24(imag_back_out4) -> fir_col_async29/24(imag_back4)
  fir_col_async30/25(real_back_out5) -> fir_col_async29/25(real_back5)
  fir_col_async30/26(imag_back_out5) -> fir_col_async29/26(imag_back5)
  fir_col_async30/27(real_back_out6) -> fir_col_async29/27(real_back6)
  fir_col_async30/28(imag_back_out6) -> fir_col_async29/28(imag_back6)
  fir_col_async30/29(real_back_out7) -> fir_col_async29/29(real_back7)
  fir_col_async30/30(imag_back_out7) -> fir_col_async29/30(imag_back7)
  fir_col_async30/31(real_back_out8) -> fir_col_async29/31(real_back8)
  fir_col_async30/32(imag_back_out8) -> fir_col_async29/32(imag_back8)
  fir_col_async31/17(real_back_out1) -> fir_col_async30/17(real_back1)
  fir_col_async31/18(imag_back_out1) -> fir_col_async30/18(imag_back1)
  fir_col_async31/19(real_back_out2) -> fir_col_async30/19(real_back2)
  fir_col_async31/20(imag_back_out2) -> fir_col_async30/20(imag_back2)
  fir_col_async31/21(real_back_out3) -> fir_col_async30/21(real_back3)
  fir_col_async31/22(imag_back_out3) -> fir_col_async30/22(imag_back3)
  fir_col_async31/23(real_back_out4) -> fir_col_async30/23(real_back4)
  fir_col_async31/24(imag_back_out4) -> fir_col_async30/24(imag_back4)
  fir_col_async31/25(real_back_out5) -> fir_col_async30/25(real_back5)
  fir_col_async31/26(imag_back_out5) -> fir_col_async30/26(imag_back5)
  fir_col_async31/27(real_back_out6) -> fir_col_async30/27(real_back6)
  fir_col_async31/28(imag_back_out6) -> fir_col_async30/28(imag_back6)
  fir_col_async31/29(real_back_out7) -> fir_col_async30/29(real_back7)
  fir_col_async31/30(imag_back_out7) -> fir_col_async30/30(imag_back7)
  fir_col_async31/31(real_back_out8) -> fir_col_async30/31(real_back8)
  fir_col_async31/32(imag_back_out8) -> fir_col_async30/32(imag_back8)
  fir_col_async32/17(real_back_out1) -> fir_col_async31/17(real_back1)
  fir_col_async32/18(imag_back_out1) -> fir_col_async31/18(imag_back1)
  fir_col_async32/19(real_back_out2) -> fir_col_async31/19(real_back2)
  fir_col_async32/20(imag_back_out2) -> fir_col_async31/20(imag_back2)
  fir_col_async32/21(real_back_out3) -> fir_col_async31/21(real_back3)
  fir_col_async32/22(imag_back_out3) -> fir_col_async31/22(imag_back3)
  fir_col_async32/23(real_back_out4) -> fir_col_async31/23(real_back4)
  fir_col_async32/24(imag_back_out4) -> fir_col_async31/24(imag_back4)
  fir_col_async32/25(real_back_out5) -> fir_col_async31/25(real_back5)
  fir_col_async32/26(imag_back_out5) -> fir_col_async31/26(imag_back5)
  fir_col_async32/27(real_back_out6) -> fir_col_async31/27(real_back6)
  fir_col_async32/28(imag_back_out6) -> fir_col_async31/28(imag_back6)
  fir_col_async32/29(real_back_out7) -> fir_col_async31/29(real_back7)
  fir_col_async32/30(imag_back_out7) -> fir_col_async31/30(imag_back7)
  fir_col_async32/31(real_back_out8) -> fir_col_async31/31(real_back8)
  fir_col_async32/32(imag_back_out8) -> fir_col_async31/32(imag_back8)
  fir_col_async32/1(real_out1) -> fir_col_async32/17(real_back1)
  fir_col_async32/2(imag_out1) -> fir_col_async32/18(imag_back1)
  fir_col_async32/3(real_out2) -> fir_col_async32/19(real_back2)
  fir_col_async32/4(imag_out2) -> fir_col_async32/20(imag_back2)
  fir_col_async32/5(real_out3) -> fir_col_async32/21(real_back3)
  fir_col_async32/6(imag_out3) -> fir_col_async32/22(imag_back3)
  fir_col_async32/7(real_out4) -> fir_col_async32/23(real_back4)
  fir_col_async32/8(imag_out4) -> fir_col_async32/24(imag_back4)
  fir_col_async32/9(real_out5) -> fir_col_async32/25(real_back5)
  fir_col_async32/10(imag_out5) -> fir_col_async32/26(imag_back5)
  fir_col_async32/11(real_out6) -> fir_col_async32/27(real_back6)
  fir_col_async32/12(imag_out6) -> fir_col_async32/28(imag_back6)
  fir_col_async32/13(real_out7) -> fir_col_async32/29(real_back7)
  fir_col_async32/14(imag_out7) -> fir_col_async32/30(imag_back7)
  fir_col_async32/15(real_out8) -> fir_col_async32/31(real_back8)
  fir_col_async32/16(imag_out8) -> fir_col_async32/32(imag_back8)
